simulink model "Simscape"  (R2021b)
(part 3 of 40)

  Transform37 : sm_lib/Frames and Transforms/Rigid Transform  TranslationMethod=Cartesian  TranslationStandardOffset=0  TranslationLengthUnit=mm  TranslationStandardAxis=+Z  TranslationCartesianOffset=smiData.RigidTransform(259).translation  TranslationROffset=0  TranslationROffsetUnits=m  TranslationZOffset=0  TranslationZOffsetUnits=m  TranslationThetaOffset=0  TranslationThetaOffsetUnits=deg  RotationMethod=ArbitraryAxis  RotationAngleUnits=rad  RotationStandardAxis=+Z  RotationAngle=smiData.RigidTransform(259).angle  RotationArbitraryAxis=smiData.RigidTransform(259).axis  FollAlignAxisA=+X  BaseAlignAxisA=+Y  FollAlignAxisB=+Y  BaseAlignAxisB=+Z  RotationSequenceAxes=FollowerAxes  RotationSequence=XYX  RotationSequenceAngles=[0 0 0]  RotationSequenceAnglesUnits=deg  RotationMatrix=[1 0 0; 0 1 0; 0 0 1]
  Transform38 : sm_lib/Frames and Transforms/Rigid Transform  TranslationMethod=Cartesian  TranslationStandardOffset=0  TranslationLengthUnit=mm  TranslationStandardAxis=+Z  TranslationCartesianOffset=smiData.RigidTransform(260).translation  TranslationROffset=0  TranslationROffsetUnits=m  TranslationZOffset=0  TranslationZOffsetUnits=m  TranslationThetaOffset=0  TranslationThetaOffsetUnits=deg  RotationMethod=ArbitraryAxis  RotationAngleUnits=rad  RotationStandardAxis=+Z  RotationAngle=smiData.RigidTransform(260).angle  RotationArbitraryAxis=smiData.RigidTransform(260).axis  FollAlignAxisA=+X  BaseAlignAxisA=+Y  FollAlignAxisB=+Y  BaseAlignAxisB=+Z  RotationSequenceAxes=FollowerAxes  RotationSequence=XYX  RotationSequenceAngles=[0 0 0]  RotationSequenceAnglesUnits=deg  RotationMatrix=[1 0 0; 0 1 0; 0 0 1]
  Transform39 : sm_lib/Frames and Transforms/Rigid Transform  TranslationMethod=Cartesian  TranslationStandardOffset=0  TranslationLengthUnit=mm  TranslationStandardAxis=+Z  TranslationCartesianOffset=smiData.RigidTransform(261).translation  TranslationROffset=0  TranslationROffsetUnits=m  TranslationZOffset=0  TranslationZOffsetUnits=m  TranslationThetaOffset=0  TranslationThetaOffsetUnits=deg  RotationMethod=ArbitraryAxis  RotationAngleUnits=rad  RotationStandardAxis=+Z  RotationAngle=smiData.RigidTransform(261).angle  RotationArbitraryAxis=smiData.RigidTransform(261).axis  FollAlignAxisA=+X  BaseAlignAxisA=+Y  FollAlignAxisB=+Y  BaseAlignAxisB=+Z  RotationSequenceAxes=FollowerAxes  RotationSequence=XYX  RotationSequenceAngles=[0 0 0]  RotationSequenceAnglesUnits=deg  RotationMatrix=[1 0 0; 0 1 0; 0 0 1]
  Transform4 : sm_lib/Frames and Transforms/Rigid Transform  TranslationMethod=Cartesian  TranslationStandardOffset=0  TranslationLengthUnit=mm  TranslationStandardAxis=+Z  TranslationCartesianOffset=smiData.RigidTransform(226).translation  TranslationROffset=0  TranslationROffsetUnits=m  TranslationZOffset=0  TranslationZOffsetUnits=m  TranslationThetaOffset=0  TranslationThetaOffsetUnits=deg  RotationMethod=ArbitraryAxis  RotationAngleUnits=rad  RotationStandardAxis=+Z  RotationAngle=smiData.RigidTransform(226).angle  RotationArbitraryAxis=smiData.RigidTransform(226).axis  FollAlignAxisA=+X  BaseAlignAxisA=+Y  FollAlignAxisB=+Y  BaseAlignAxisB=+Z  RotationSequenceAxes=FollowerAxes  RotationSequence=XYX  RotationSequenceAngles=[0 0 0]  RotationSequenceAnglesUnits=deg  RotationMatrix=[1 0 0; 0 1 0; 0 0 1]
  Transform40 : sm_lib/Frames and Transforms/Rigid Transform  TranslationMethod=Cartesian  TranslationStandardOffset=0  TranslationLengthUnit=mm  TranslationStandardAxis=+Z  TranslationCartesianOffset=smiData.RigidTransform(262).translation  TranslationROffset=0  TranslationROffsetUnits=m  TranslationZOffset=0  TranslationZOffsetUnits=m  TranslationThetaOffset=0  TranslationThetaOffsetUnits=deg  RotationMethod=ArbitraryAxis  RotationAngleUnits=rad  RotationStandardAxis=+Z  RotationAngle=smiData.RigidTransform(262).angle  RotationArbitraryAxis=smiData.RigidTransform(262).axis  FollAlignAxisA=+X  BaseAlignAxisA=+Y  FollAlignAxisB=+Y  BaseAlignAxisB=+Z  RotationSequenceAxes=FollowerAxes  RotationSequence=XYX  RotationSequenceAngles=[0 0 0]  RotationSequenceAnglesUnits=deg  RotationMatrix=[1 0 0; 0 1 0; 0 0 1]
  Transform41 : sm_lib/Frames and Transforms/Rigid Transform  TranslationMethod=Cartesian  TranslationStandardOffset=0  TranslationLengthUnit=mm  TranslationStandardAxis=+Z  TranslationCartesianOffset=smiData.RigidTransform(263).translation  TranslationROffset=0  TranslationROffsetUnits=m  TranslationZOffset=0  TranslationZOffsetUnits=m  TranslationThetaOffset=0  TranslationThetaOffsetUnits=deg  RotationMethod=ArbitraryAxis  RotationAngleUnits=rad  RotationStandardAxis=+Z  RotationAngle=smiData.RigidTransform(263).angle  RotationArbitraryAxis=smiData.RigidTransform(263).axis  FollAlignAxisA=+X  BaseAlignAxisA=+Y  FollAlignAxisB=+Y  BaseAlignAxisB=+Z  RotationSequenceAxes=FollowerAxes  RotationSequence=XYX  RotationSequenceAngles=[0 0 0]  RotationSequenceAnglesUnits=deg  RotationMatrix=[1 0 0; 0 1 0; 0 0 1]
  Transform42 : sm_lib/Frames and Transforms/Rigid Transform  TranslationMethod=Cartesian  TranslationStandardOffset=0  TranslationLengthUnit=mm  TranslationStandardAxis=+Z  TranslationCartesianOffset=smiData.RigidTransform(264).translation  TranslationROffset=0  TranslationROffsetUnits=m  TranslationZOffset=0  TranslationZOffsetUnits=m  TranslationThetaOffset=0  TranslationThetaOffsetUnits=deg  RotationMethod=ArbitraryAxis  RotationAngleUnits=rad  RotationStandardAxis=+Z  RotationAngle=smiData.RigidTransform(264).angle  RotationArbitraryAxis=smiData.RigidTransform(264).axis  FollAlignAxisA=+X  BaseAlignAxisA=+Y  FollAlignAxisB=+Y  BaseAlignAxisB=+Z  RotationSequenceAxes=FollowerAxes  RotationSequence=XYX  RotationSequenceAngles=[0 0 0]  RotationSequenceAnglesUnits=deg  RotationMatrix=[1 0 0; 0 1 0; 0 0 1]
  Transform43 : sm_lib/Frames and Transforms/Rigid Transform  TranslationMethod=Cartesian  TranslationStandardOffset=0  TranslationLengthUnit=mm  TranslationStandardAxis=+Z  TranslationCartesianOffset=smiData.RigidTransform(265).translation  TranslationROffset=0  TranslationROffsetUnits=m  TranslationZOffset=0  TranslationZOffsetUnits=m  TranslationThetaOffset=0  TranslationThetaOffsetUnits=deg  RotationMethod=ArbitraryAxis  RotationAngleUnits=rad  RotationStandardAxis=+Z  RotationAngle=smiData.RigidTransform(265).angle  RotationArbitraryAxis=smiData.RigidTransform(265).axis  FollAlignAxisA=+X  BaseAlignAxisA=+Y  FollAlignAxisB=+Y  BaseAlignAxisB=+Z  RotationSequenceAxes=FollowerAxes  RotationSequence=XYX  RotationSequenceAngles=[0 0 0]  RotationSequenceAnglesUnits=deg  RotationMatrix=[1 0 0; 0 1 0; 0 0 1]
  Transform44 : sm_lib/Frames and Transforms/Rigid Transform  TranslationMethod=Cartesian  TranslationStandardOffset=0  TranslationLengthUnit=mm  TranslationStandardAxis=+Z  TranslationCartesianOffset=smiData.RigidTransform(266).translation  TranslationROffset=0  TranslationROffsetUnits=m  TranslationZOffset=0  TranslationZOffsetUnits=m  TranslationThetaOffset=0  TranslationThetaOffsetUnits=deg  RotationMethod=ArbitraryAxis  RotationAngleUnits=rad  RotationStandardAxis=+Z  RotationAngle=smiData.RigidTransform(266).angle  RotationArbitraryAxis=smiData.RigidTransform(266).axis  FollAlignAxisA=+X  BaseAlignAxisA=+Y  FollAlignAxisB=+Y  BaseAlignAxisB=+Z  RotationSequenceAxes=FollowerAxes  RotationSequence=XYX  RotationSequenceAngles=[0 0 0]  RotationSequenceAnglesUnits=deg  RotationMatrix=[1 0 0; 0 1 0; 0 0 1]
  Transform45 : sm_lib/Frames and Transforms/Rigid Transform  TranslationMethod=Cartesian  TranslationStandardOffset=0  TranslationLengthUnit=mm  TranslationStandardAxis=+Z  TranslationCartesianOffset=smiData.RigidTransform(267).translation  TranslationROffset=0  TranslationROffsetUnits=m  TranslationZOffset=0  TranslationZOffsetUnits=m  TranslationThetaOffset=0  TranslationThetaOffsetUnits=deg  RotationMethod=ArbitraryAxis  RotationAngleUnits=rad  RotationStandardAxis=+Z  RotationAngle=smiData.RigidTransform(267).angle  RotationArbitraryAxis=smiData.RigidTransform(267).axis  FollAlignAxisA=+X  BaseAlignAxisA=+Y  FollAlignAxisB=+Y  BaseAlignAxisB=+Z  RotationSequenceAxes=FollowerAxes  RotationSequence=XYX  RotationSequenceAngles=[0 0 0]  RotationSequenceAnglesUnits=deg  RotationMatrix=[1 0 0; 0 1 0; 0 0 1]
  Transform46 : sm_lib/Frames and Transforms/Rigid Transform  TranslationMethod=Cartesian  TranslationStandardOffset=0  TranslationLengthUnit=mm  TranslationStandardAxis=+Z  TranslationCartesianOffset=smiData.RigidTransform(268).translation  TranslationROffset=0  TranslationROffsetUnits=m  TranslationZOffset=0  TranslationZOffsetUnits=m  TranslationThetaOffset=0  TranslationThetaOffsetUnits=deg  RotationMethod=ArbitraryAxis  RotationAngleUnits=rad  RotationStandardAxis=+Z  RotationAngle=smiData.RigidTransform(268).angle  RotationArbitraryAxis=smiData.RigidTransform(268).axis  FollAlignAxisA=+X  BaseAlignAxisA=+Y  FollAlignAxisB=+Y  BaseAlignAxisB=+Z  RotationSequenceAxes=FollowerAxes  RotationSequence=XYX  RotationSequenceAngles=[0 0 0]  RotationSequenceAnglesUnits=deg  RotationMatrix=[1 0 0; 0 1 0; 0 0 1]
  Transform47 : sm_lib/Frames and Transforms/Rigid Transform  TranslationMethod=Cartesian  TranslationStandardOffset=0  TranslationLengthUnit=mm  TranslationStandardAxis=+Z  TranslationCartesianOffset=smiData.RigidTransform(269).translation  TranslationROffset=0  TranslationROffsetUnits=m  TranslationZOffset=0  TranslationZOffsetUnits=m  TranslationThetaOffset=0  TranslationThetaOffsetUnits=deg  RotationMethod=ArbitraryAxis  RotationAngleUnits=rad  RotationStandardAxis=+Z  RotationAngle=smiData.RigidTransform(269).angle  RotationArbitraryAxis=smiData.RigidTransform(269).axis  FollAlignAxisA=+X  BaseAlignAxisA=+Y  FollAlignAxisB=+Y  BaseAlignAxisB=+Z  RotationSequenceAxes=FollowerAxes  RotationSequence=XYX  RotationSequenceAngles=[0 0 0]  RotationSequenceAnglesUnits=deg  RotationMatrix=[1 0 0; 0 1 0; 0 0 1]
  Transform48 : sm_lib/Frames and Transforms/Rigid Transform  TranslationMethod=Cartesian  TranslationStandardOffset=0  TranslationLengthUnit=mm  TranslationStandardAxis=+Z  TranslationCartesianOffset=smiData.RigidTransform(270).translation  TranslationROffset=0  TranslationROffsetUnits=m  TranslationZOffset=0  TranslationZOffsetUnits=m  TranslationThetaOffset=0  TranslationThetaOffsetUnits=deg  RotationMethod=ArbitraryAxis  RotationAngleUnits=rad  RotationStandardAxis=+Z  RotationAngle=smiData.RigidTransform(270).angle  RotationArbitraryAxis=smiData.RigidTransform(270).axis  FollAlignAxisA=+X  BaseAlignAxisA=+Y  FollAlignAxisB=+Y  BaseAlignAxisB=+Z  RotationSequenceAxes=FollowerAxes  RotationSequence=XYX  RotationSequenceAngles=[0 0 0]  RotationSequenceAnglesUnits=deg  RotationMatrix=[1 0 0; 0 1 0; 0 0 1]
  Transform49 : sm_lib/Frames and Transforms/Rigid Transform  TranslationMethod=Cartesian  TranslationStandardOffset=0  TranslationLengthUnit=mm  TranslationStandardAxis=+Z  TranslationCartesianOffset=smiData.RigidTransform(271).translation  TranslationROffset=0  TranslationROffsetUnits=m  TranslationZOffset=0  TranslationZOffsetUnits=m  TranslationThetaOffset=0  TranslationThetaOffsetUnits=deg  RotationMethod=ArbitraryAxis  RotationAngleUnits=rad  RotationStandardAxis=+Z  RotationAngle=smiData.RigidTransform(271).angle  RotationArbitraryAxis=smiData.RigidTransform(271).axis  FollAlignAxisA=+X  BaseAlignAxisA=+Y  FollAlignAxisB=+Y  BaseAlignAxisB=+Z  RotationSequenceAxes=FollowerAxes  RotationSequence=XYX  RotationSequenceAngles=[0 0 0]  RotationSequenceAnglesUnits=deg  RotationMatrix=[1 0 0; 0 1 0; 0 0 1]
  Transform5 : sm_lib/Frames and Transforms/Rigid Transform  TranslationMethod=Cartesian  TranslationStandardOffset=0  TranslationLengthUnit=mm  TranslationStandardAxis=+Z  TranslationCartesianOffset=smiData.RigidTransform(227).translation  TranslationROffset=0  TranslationROffsetUnits=m  TranslationZOffset=0  TranslationZOffsetUnits=m  TranslationThetaOffset=0  TranslationThetaOffsetUnits=deg  RotationMethod=ArbitraryAxis  RotationAngleUnits=rad  RotationStandardAxis=+Z  RotationAngle=smiData.RigidTransform(227).angle  RotationArbitraryAxis=smiData.RigidTransform(227).axis  FollAlignAxisA=+X  BaseAlignAxisA=+Y  FollAlignAxisB=+Y  BaseAlignAxisB=+Z  RotationSequenceAxes=FollowerAxes  RotationSequence=XYX  RotationSequenceAngles=[0 0 0]  RotationSequenceAnglesUnits=deg  RotationMatrix=[1 0 0; 0 1 0; 0 0 1]
  Transform50 : sm_lib/Frames and Transforms/Rigid Transform  TranslationMethod=Cartesian  TranslationStandardOffset=0  TranslationLengthUnit=mm  TranslationStandardAxis=+Z  TranslationCartesianOffset=smiData.RigidTransform(272).translation  TranslationROffset=0  TranslationROffsetUnits=m  TranslationZOffset=0  TranslationZOffsetUnits=m  TranslationThetaOffset=0  TranslationThetaOffsetUnits=deg  RotationMethod=ArbitraryAxis  RotationAngleUnits=rad  RotationStandardAxis=+Z  RotationAngle=smiData.RigidTransform(272).angle  RotationArbitraryAxis=smiData.RigidTransform(272).axis  FollAlignAxisA=+X  BaseAlignAxisA=+Y  FollAlignAxisB=+Y  BaseAlignAxisB=+Z  RotationSequenceAxes=FollowerAxes  RotationSequence=XYX  RotationSequenceAngles=[0 0 0]  RotationSequenceAnglesUnits=deg  RotationMatrix=[1 0 0; 0 1 0; 0 0 1]
  Transform51 : sm_lib/Frames and Transforms/Rigid Transform  TranslationMethod=Cartesian  TranslationStandardOffset=0  TranslationLengthUnit=mm  TranslationStandardAxis=+Z  TranslationCartesianOffset=smiData.RigidTransform(273).translation  TranslationROffset=0  TranslationROffsetUnits=m  TranslationZOffset=0  TranslationZOffsetUnits=m  TranslationThetaOffset=0  TranslationThetaOffsetUnits=deg  RotationMethod=ArbitraryAxis  RotationAngleUnits=rad  RotationStandardAxis=+Z  RotationAngle=smiData.RigidTransform(273).angle  RotationArbitraryAxis=smiData.RigidTransform(273).axis  FollAlignAxisA=+X  BaseAlignAxisA=+Y  FollAlignAxisB=+Y  BaseAlignAxisB=+Z  RotationSequenceAxes=FollowerAxes  RotationSequence=XYX  RotationSequenceAngles=[0 0 0]  RotationSequenceAnglesUnits=deg  RotationMatrix=[1 0 0; 0 1 0; 0 0 1]
  Transform52 : sm_lib/Frames and Transforms/Rigid Transform  TranslationMethod=Cartesian  TranslationStandardOffset=0  TranslationLengthUnit=mm  TranslationStandardAxis=+Z  TranslationCartesianOffset=smiData.RigidTransform(274).translation  TranslationROffset=0  TranslationROffsetUnits=m  TranslationZOffset=0  TranslationZOffsetUnits=m  TranslationThetaOffset=0  TranslationThetaOffsetUnits=deg  RotationMethod=ArbitraryAxis  RotationAngleUnits=rad  RotationStandardAxis=+Z  RotationAngle=smiData.RigidTransform(274).angle  RotationArbitraryAxis=smiData.RigidTransform(274).axis  FollAlignAxisA=+X  BaseAlignAxisA=+Y  FollAlignAxisB=+Y  BaseAlignAxisB=+Z  RotationSequenceAxes=FollowerAxes  RotationSequence=XYX  RotationSequenceAngles=[0 0 0]  RotationSequenceAnglesUnits=deg  RotationMatrix=[1 0 0; 0 1 0; 0 0 1]
  Transform53 : sm_lib/Frames and Transforms/Rigid Transform  TranslationMethod=Cartesian  TranslationStandardOffset=0  TranslationLengthUnit=mm  TranslationStandardAxis=+Z  TranslationCartesianOffset=smiData.RigidTransform(275).translation  TranslationROffset=0  TranslationROffsetUnits=m  TranslationZOffset=0  TranslationZOffsetUnits=m  TranslationThetaOffset=0  TranslationThetaOffsetUnits=deg  RotationMethod=ArbitraryAxis  RotationAngleUnits=rad  RotationStandardAxis=+Z  RotationAngle=smiData.RigidTransform(275).angle  RotationArbitraryAxis=smiData.RigidTransform(275).axis  FollAlignAxisA=+X  BaseAlignAxisA=+Y  FollAlignAxisB=+Y  BaseAlignAxisB=+Z  RotationSequenceAxes=FollowerAxes  RotationSequence=XYX  RotationSequenceAngles=[0 0 0]  RotationSequenceAnglesUnits=deg  RotationMatrix=[1 0 0; 0 1 0; 0 0 1]
  Transform54 : sm_lib/Frames and Transforms/Rigid Transform  TranslationMethod=Cartesian  TranslationStandardOffset=0  TranslationLengthUnit=mm  TranslationStandardAxis=+Z  TranslationCartesianOffset=smiData.RigidTransform(276).translation  TranslationROffset=0  TranslationROffsetUnits=m  TranslationZOffset=0  TranslationZOffsetUnits=m  TranslationThetaOffset=0  TranslationThetaOffsetUnits=deg  RotationMethod=ArbitraryAxis  RotationAngleUnits=rad  RotationStandardAxis=+Z  RotationAngle=smiData.RigidTransform(276).angle  RotationArbitraryAxis=smiData.RigidTransform(276).axis  FollAlignAxisA=+X  BaseAlignAxisA=+Y  FollAlignAxisB=+Y  BaseAlignAxisB=+Z  RotationSequenceAxes=FollowerAxes  RotationSequence=XYX  RotationSequenceAngles=[0 0 0]  RotationSequenceAnglesUnits=deg  RotationMatrix=[1 0 0; 0 1 0; 0 0 1]
  Transform55 : sm_lib/Frames and Transforms/Rigid Transform  TranslationMethod=Cartesian  TranslationStandardOffset=0  TranslationLengthUnit=mm  TranslationStandardAxis=+Z  TranslationCartesianOffset=smiData.RigidTransform(277).translation  TranslationROffset=0  TranslationROffsetUnits=m  TranslationZOffset=0  TranslationZOffsetUnits=m  TranslationThetaOffset=0  TranslationThetaOffsetUnits=deg  RotationMethod=ArbitraryAxis  RotationAngleUnits=rad  RotationStandardAxis=+Z  RotationAngle=smiData.RigidTransform(277).angle  RotationArbitraryAxis=smiData.RigidTransform(277).axis  FollAlignAxisA=+X  BaseAlignAxisA=+Y  FollAlignAxisB=+Y  BaseAlignAxisB=+Z  RotationSequenceAxes=FollowerAxes  RotationSequence=XYX  RotationSequenceAngles=[0 0 0]  RotationSequenceAnglesUnits=deg  RotationMatrix=[1 0 0; 0 1 0; 0 0 1]
  Transform56 : sm_lib/Frames and Transforms/Rigid Transform  TranslationMethod=Cartesian  TranslationStandardOffset=0  TranslationLengthUnit=mm  TranslationStandardAxis=+Z  TranslationCartesianOffset=smiData.RigidTransform(278).translation  TranslationROffset=0  TranslationROffsetUnits=m  TranslationZOffset=0  TranslationZOffsetUnits=m  TranslationThetaOffset=0  TranslationThetaOffsetUnits=deg  RotationMethod=ArbitraryAxis  RotationAngleUnits=rad  RotationStandardAxis=+Z  RotationAngle=smiData.RigidTransform(278).angle  RotationArbitraryAxis=smiData.RigidTransform(278).axis  FollAlignAxisA=+X  BaseAlignAxisA=+Y  FollAlignAxisB=+Y  BaseAlignAxisB=+Z  RotationSequenceAxes=FollowerAxes  RotationSequence=XYX  RotationSequenceAngles=[0 0 0]  RotationSequenceAnglesUnits=deg  RotationMatrix=[1 0 0; 0 1 0; 0 0 1]
  Transform57 : sm_lib/Frames and Transforms/Rigid Transform  TranslationMethod=Cartesian  TranslationStandardOffset=0  TranslationLengthUnit=mm  TranslationStandardAxis=+Z  TranslationCartesianOffset=smiData.RigidTransform(279).translation  TranslationROffset=0  TranslationROffsetUnits=m  TranslationZOffset=0  TranslationZOffsetUnits=m  TranslationThetaOffset=0  TranslationThetaOffsetUnits=deg  RotationMethod=ArbitraryAxis  RotationAngleUnits=rad  RotationStandardAxis=+Z  RotationAngle=smiData.RigidTransform(279).angle  RotationArbitraryAxis=smiData.RigidTransform(279).axis  FollAlignAxisA=+X  BaseAlignAxisA=+Y  FollAlignAxisB=+Y  BaseAlignAxisB=+Z  RotationSequenceAxes=FollowerAxes  RotationSequence=XYX  RotationSequenceAngles=[0 0 0]  RotationSequenceAnglesUnits=deg  RotationMatrix=[1 0 0; 0 1 0; 0 0 1]
  Transform58 : sm_lib/Frames and Transforms/Rigid Transform  TranslationMethod=Cartesian  TranslationStandardOffset=0  TranslationLengthUnit=mm  TranslationStandardAxis=+Z  TranslationCartesianOffset=smiData.RigidTransform(280).translation  TranslationROffset=0  TranslationROffsetUnits=m  TranslationZOffset=0  TranslationZOffsetUnits=m  TranslationThetaOffset=0  TranslationThetaOffsetUnits=deg  RotationMethod=ArbitraryAxis  RotationAngleUnits=rad  RotationStandardAxis=+Z  RotationAngle=smiData.RigidTransform(280).angle  RotationArbitraryAxis=smiData.RigidTransform(280).axis  FollAlignAxisA=+X  BaseAlignAxisA=+Y  FollAlignAxisB=+Y  BaseAlignAxisB=+Z  RotationSequenceAxes=FollowerAxes  RotationSequence=XYX  RotationSequenceAngles=[0 0 0]  RotationSequenceAnglesUnits=deg  RotationMatrix=[1 0 0; 0 1 0; 0 0 1]
  Transform59 : sm_lib/Frames and Transforms/Rigid Transform  TranslationMethod=Cartesian  TranslationStandardOffset=0  TranslationLengthUnit=mm  TranslationStandardAxis=+Z  TranslationCartesianOffset=smiData.RigidTransform(281).translation  TranslationROffset=0  TranslationROffsetUnits=m  TranslationZOffset=0  TranslationZOffsetUnits=m  TranslationThetaOffset=0  TranslationThetaOffsetUnits=deg  RotationMethod=ArbitraryAxis  RotationAngleUnits=rad  RotationStandardAxis=+Z  RotationAngle=smiData.RigidTransform(281).angle  RotationArbitraryAxis=smiData.RigidTransform(281).axis  FollAlignAxisA=+X  BaseAlignAxisA=+Y  FollAlignAxisB=+Y  BaseAlignAxisB=+Z  RotationSequenceAxes=FollowerAxes  RotationSequence=XYX  RotationSequenceAngles=[0 0 0]  RotationSequenceAnglesUnits=deg  RotationMatrix=[1 0 0; 0 1 0; 0 0 1]
  Transform6 : sm_lib/Frames and Transforms/Rigid Transform  TranslationMethod=Cartesian  TranslationStandardOffset=0  TranslationLengthUnit=mm  TranslationStandardAxis=+Z  TranslationCartesianOffset=smiData.RigidTransform(228).translation  TranslationROffset=0  TranslationROffsetUnits=m  TranslationZOffset=0  TranslationZOffsetUnits=m  TranslationThetaOffset=0  TranslationThetaOffsetUnits=deg  RotationMethod=ArbitraryAxis  RotationAngleUnits=rad  RotationStandardAxis=+Z  RotationAngle=smiData.RigidTransform(228).angle  RotationArbitraryAxis=smiData.RigidTransform(228).axis  FollAlignAxisA=+X  BaseAlignAxisA=+Y  FollAlignAxisB=+Y  BaseAlignAxisB=+Z  RotationSequenceAxes=FollowerAxes  RotationSequence=XYX  RotationSequenceAngles=[0 0 0]  RotationSequenceAnglesUnits=deg  RotationMatrix=[1 0 0; 0 1 0; 0 0 1]
  Transform60 : sm_lib/Frames and Transforms/Rigid Transform  TranslationMethod=Cartesian  TranslationStandardOffset=0  TranslationLengthUnit=mm  TranslationStandardAxis=+Z  TranslationCartesianOffset=smiData.RigidTransform(282).translation  TranslationROffset=0  TranslationROffsetUnits=m  TranslationZOffset=0  TranslationZOffsetUnits=m  TranslationThetaOffset=0  TranslationThetaOffsetUnits=deg  RotationMethod=ArbitraryAxis  RotationAngleUnits=rad  RotationStandardAxis=+Z  RotationAngle=smiData.RigidTransform(282).angle  RotationArbitraryAxis=smiData.RigidTransform(282).axis  FollAlignAxisA=+X  BaseAlignAxisA=+Y  FollAlignAxisB=+Y  BaseAlignAxisB=+Z  RotationSequenceAxes=FollowerAxes  RotationSequence=XYX  RotationSequenceAngles=[0 0 0]  RotationSequenceAnglesUnits=deg  RotationMatrix=[1 0 0; 0 1 0; 0 0 1]
  Transform61 : sm_lib/Frames and Transforms/Rigid Transform  TranslationMethod=Cartesian  TranslationStandardOffset=0  TranslationLengthUnit=mm  TranslationStandardAxis=+Z  TranslationCartesianOffset=smiData.RigidTransform(283).translation  TranslationROffset=0  TranslationROffsetUnits=m  TranslationZOffset=0  TranslationZOffsetUnits=m  TranslationThetaOffset=0  TranslationThetaOffsetUnits=deg  RotationMethod=ArbitraryAxis  RotationAngleUnits=rad  RotationStandardAxis=+Z  RotationAngle=smiData.RigidTransform(283).angle  RotationArbitraryAxis=smiData.RigidTransform(283).axis  FollAlignAxisA=+X  BaseAlignAxisA=+Y  FollAlignAxisB=+Y  BaseAlignAxisB=+Z  RotationSequenceAxes=FollowerAxes  RotationSequence=XYX  RotationSequenceAngles=[0 0 0]  RotationSequenceAnglesUnits=deg  RotationMatrix=[1 0 0; 0 1 0; 0 0 1]
  Transform62 : sm_lib/Frames and Transforms/Rigid Transform  TranslationMethod=Cartesian  TranslationStandardOffset=0  TranslationLengthUnit=mm  TranslationStandardAxis=+Z  TranslationCartesianOffset=smiData.RigidTransform(284).translation  TranslationROffset=0  TranslationROffsetUnits=m  TranslationZOffset=0  TranslationZOffsetUnits=m  TranslationThetaOffset=0  TranslationThetaOffsetUnits=deg  RotationMethod=ArbitraryAxis  RotationAngleUnits=rad  RotationStandardAxis=+Z  RotationAngle=smiData.RigidTransform(284).angle  RotationArbitraryAxis=smiData.RigidTransform(284).axis  FollAlignAxisA=+X  BaseAlignAxisA=+Y  FollAlignAxisB=+Y  BaseAlignAxisB=+Z  RotationSequenceAxes=FollowerAxes  RotationSequence=XYX  RotationSequenceAngles=[0 0 0]  RotationSequenceAnglesUnits=deg  RotationMatrix=[1 0 0; 0 1 0; 0 0 1]
  Transform63 : sm_lib/Frames and Transforms/Rigid Transform  TranslationMethod=Cartesian  TranslationStandardOffset=0  TranslationLengthUnit=mm  TranslationStandardAxis=+Z  TranslationCartesianOffset=smiData.RigidTransform(285).translation  TranslationROffset=0  TranslationROffsetUnits=m  TranslationZOffset=0  TranslationZOffsetUnits=m  TranslationThetaOffset=0  TranslationThetaOffsetUnits=deg  RotationMethod=ArbitraryAxis  RotationAngleUnits=rad  RotationStandardAxis=+Z  RotationAngle=smiData.RigidTransform(285).angle  RotationArbitraryAxis=smiData.RigidTransform(285).axis  FollAlignAxisA=+X  BaseAlignAxisA=+Y  FollAlignAxisB=+Y  BaseAlignAxisB=+Z  RotationSequenceAxes=FollowerAxes  RotationSequence=XYX  RotationSequenceAngles=[0 0 0]  RotationSequenceAnglesUnits=deg  RotationMatrix=[1 0 0; 0 1 0; 0 0 1]
  Transform64 : sm_lib/Frames and Transforms/Rigid Transform  TranslationMethod=Cartesian  TranslationStandardOffset=0  TranslationLengthUnit=mm  TranslationStandardAxis=+Z  TranslationCartesianOffset=smiData.RigidTransform(286).translation  TranslationROffset=0  TranslationROffsetUnits=m  TranslationZOffset=0  TranslationZOffsetUnits=m  TranslationThetaOffset=0  TranslationThetaOffsetUnits=deg  RotationMethod=ArbitraryAxis  RotationAngleUnits=rad  RotationStandardAxis=+Z  RotationAngle=smiData.RigidTransform(286).angle  RotationArbitraryAxis=smiData.RigidTransform(286).axis  FollAlignAxisA=+X  BaseAlignAxisA=+Y  FollAlignAxisB=+Y  BaseAlignAxisB=+Z  RotationSequenceAxes=FollowerAxes  RotationSequence=XYX  RotationSequenceAngles=[0 0 0]  RotationSequenceAnglesUnits=deg  RotationMatrix=[1 0 0; 0 1 0; 0 0 1]
  Transform65 : sm_lib/Frames and Transforms/Rigid Transform  TranslationMethod=Cartesian  TranslationStandardOffset=0  TranslationLengthUnit=mm  TranslationStandardAxis=+Z  TranslationCartesianOffset=smiData.RigidTransform(287).translation  TranslationROffset=0  TranslationROffsetUnits=m  TranslationZOffset=0  TranslationZOffsetUnits=m  TranslationThetaOffset=0  TranslationThetaOffsetUnits=deg  RotationMethod=ArbitraryAxis  RotationAngleUnits=rad  RotationStandardAxis=+Z  RotationAngle=smiData.RigidTransform(287).angle  RotationArbitraryAxis=smiData.RigidTransform(287).axis  FollAlignAxisA=+X  BaseAlignAxisA=+Y  FollAlignAxisB=+Y  BaseAlignAxisB=+Z  RotationSequenceAxes=FollowerAxes  RotationSequence=XYX  RotationSequenceAngles=[0 0 0]  RotationSequenceAnglesUnits=deg  RotationMatrix=[1 0 0; 0 1 0; 0 0 1]
  Transform66 : sm_lib/Frames and Transforms/Rigid Transform  TranslationMethod=Cartesian  TranslationStandardOffset=0  TranslationLengthUnit=mm  TranslationStandardAxis=+Z  TranslationCartesianOffset=smiData.RigidTransform(288).translation  TranslationROffset=0  TranslationROffsetUnits=m  TranslationZOffset=0  TranslationZOffsetUnits=m  TranslationThetaOffset=0  TranslationThetaOffsetUnits=deg  RotationMethod=ArbitraryAxis  RotationAngleUnits=rad  RotationStandardAxis=+Z  RotationAngle=smiData.RigidTransform(288).angle  RotationArbitraryAxis=smiData.RigidTransform(288).axis  FollAlignAxisA=+X  BaseAlignAxisA=+Y  FollAlignAxisB=+Y  BaseAlignAxisB=+Z  RotationSequenceAxes=FollowerAxes  RotationSequence=XYX  RotationSequenceAngles=[0 0 0]  RotationSequenceAnglesUnits=deg  RotationMatrix=[1 0 0; 0 1 0; 0 0 1]
  Transform67 : sm_lib/Frames and Transforms/Rigid Transform  TranslationMethod=Cartesian  TranslationStandardOffset=0  TranslationLengthUnit=mm  TranslationStandardAxis=+Z  TranslationCartesianOffset=smiData.RigidTransform(289).translation  TranslationROffset=0  TranslationROffsetUnits=m  TranslationZOffset=0  TranslationZOffsetUnits=m  TranslationThetaOffset=0  TranslationThetaOffsetUnits=deg  RotationMethod=ArbitraryAxis  RotationAngleUnits=rad  RotationStandardAxis=+Z  RotationAngle=smiData.RigidTransform(289).angle  RotationArbitraryAxis=smiData.RigidTransform(289).axis  FollAlignAxisA=+X  BaseAlignAxisA=+Y  FollAlignAxisB=+Y  BaseAlignAxisB=+Z  RotationSequenceAxes=FollowerAxes  RotationSequence=XYX  RotationSequenceAngles=[0 0 0]  RotationSequenceAnglesUnits=deg  RotationMatrix=[1 0 0; 0 1 0; 0 0 1]
  Transform68 : sm_lib/Frames and Transforms/Rigid Transform  TranslationMethod=Cartesian  TranslationStandardOffset=0  TranslationLengthUnit=mm  TranslationStandardAxis=+Z  TranslationCartesianOffset=smiData.RigidTransform(290).translation  TranslationROffset=0  TranslationROffsetUnits=m  TranslationZOffset=0  TranslationZOffsetUnits=m  TranslationThetaOffset=0  TranslationThetaOffsetUnits=deg  RotationMethod=ArbitraryAxis  RotationAngleUnits=rad  RotationStandardAxis=+Z  RotationAngle=smiData.RigidTransform(290).angle  RotationArbitraryAxis=smiData.RigidTransform(290).axis  FollAlignAxisA=+X  BaseAlignAxisA=+Y  FollAlignAxisB=+Y  BaseAlignAxisB=+Z  RotationSequenceAxes=FollowerAxes  RotationSequence=XYX  RotationSequenceAngles=[0 0 0]  RotationSequenceAnglesUnits=deg  RotationMatrix=[1 0 0; 0 1 0; 0 0 1]
  Transform69 : sm_lib/Frames and Transforms/Rigid Transform  TranslationMethod=Cartesian  TranslationStandardOffset=0  TranslationLengthUnit=mm  TranslationStandardAxis=+Z  TranslationCartesianOffset=smiData.RigidTransform(291).translation  TranslationROffset=0  TranslationROffsetUnits=m  TranslationZOffset=0  TranslationZOffsetUnits=m  TranslationThetaOffset=0  TranslationThetaOffsetUnits=deg  RotationMethod=ArbitraryAxis  RotationAngleUnits=rad  RotationStandardAxis=+Z  RotationAngle=smiData.RigidTransform(291).angle  RotationArbitraryAxis=smiData.RigidTransform(291).axis  FollAlignAxisA=+X  BaseAlignAxisA=+Y  FollAlignAxisB=+Y  BaseAlignAxisB=+Z  RotationSequenceAxes=FollowerAxes  RotationSequence=XYX  RotationSequenceAngles=[0 0 0]  RotationSequenceAnglesUnits=deg  RotationMatrix=[1 0 0; 0 1 0; 0 0 1]
  Transform7 : sm_lib/Frames and Transforms/Rigid Transform  TranslationMethod=Cartesian  TranslationStandardOffset=0  TranslationLengthUnit=mm  TranslationStandardAxis=+Z  TranslationCartesianOffset=smiData.RigidTransform(229).translation  TranslationROffset=0  TranslationROffsetUnits=m  TranslationZOffset=0  TranslationZOffsetUnits=m  TranslationThetaOffset=0  TranslationThetaOffsetUnits=deg  RotationMethod=ArbitraryAxis  RotationAngleUnits=rad  RotationStandardAxis=+Z  RotationAngle=smiData.RigidTransform(229).angle  RotationArbitraryAxis=smiData.RigidTransform(229).axis  FollAlignAxisA=+X  BaseAlignAxisA=+Y  FollAlignAxisB=+Y  BaseAlignAxisB=+Z  RotationSequenceAxes=FollowerAxes  RotationSequence=XYX  RotationSequenceAngles=[0 0 0]  RotationSequenceAnglesUnits=deg  RotationMatrix=[1 0 0; 0 1 0; 0 0 1]
  Transform70 : sm_lib/Frames and Transforms/Rigid Transform  TranslationMethod=Cartesian  TranslationStandardOffset=0  TranslationLengthUnit=mm  TranslationStandardAxis=+Z  TranslationCartesianOffset=smiData.RigidTransform(292).translation  TranslationROffset=0  TranslationROffsetUnits=m  TranslationZOffset=0  TranslationZOffsetUnits=m  TranslationThetaOffset=0  TranslationThetaOffsetUnits=deg  RotationMethod=ArbitraryAxis  RotationAngleUnits=rad  RotationStandardAxis=+Z  RotationAngle=smiData.RigidTransform(292).angle  RotationArbitraryAxis=smiData.RigidTransform(292).axis  FollAlignAxisA=+X  BaseAlignAxisA=+Y  FollAlignAxisB=+Y  BaseAlignAxisB=+Z  RotationSequenceAxes=FollowerAxes  RotationSequence=XYX  RotationSequenceAngles=[0 0 0]  RotationSequenceAnglesUnits=deg  RotationMatrix=[1 0 0; 0 1 0; 0 0 1]
  Transform71 : sm_lib/Frames and Transforms/Rigid Transform  TranslationMethod=Cartesian  TranslationStandardOffset=0  TranslationLengthUnit=mm  TranslationStandardAxis=+Z  TranslationCartesianOffset=smiData.RigidTransform(293).translation  TranslationROffset=0  TranslationROffsetUnits=m  TranslationZOffset=0  TranslationZOffsetUnits=m  TranslationThetaOffset=0  TranslationThetaOffsetUnits=deg  RotationMethod=ArbitraryAxis  RotationAngleUnits=rad  RotationStandardAxis=+Z  RotationAngle=smiData.RigidTransform(293).angle  RotationArbitraryAxis=smiData.RigidTransform(293).axis  FollAlignAxisA=+X  BaseAlignAxisA=+Y  FollAlignAxisB=+Y  BaseAlignAxisB=+Z  RotationSequenceAxes=FollowerAxes  RotationSequence=XYX  RotationSequenceAngles=[0 0 0]  RotationSequenceAnglesUnits=deg  RotationMatrix=[1 0 0; 0 1 0; 0 0 1]
  Transform72 : sm_lib/Frames and Transforms/Rigid Transform  TranslationMethod=Cartesian  TranslationStandardOffset=0  TranslationLengthUnit=mm  TranslationStandardAxis=+Z  TranslationCartesianOffset=smiData.RigidTransform(294).translation  TranslationROffset=0  TranslationROffsetUnits=m  TranslationZOffset=0  TranslationZOffsetUnits=m  TranslationThetaOffset=0  TranslationThetaOffsetUnits=deg  RotationMethod=ArbitraryAxis  RotationAngleUnits=rad  RotationStandardAxis=+Z  RotationAngle=smiData.RigidTransform(294).angle  RotationArbitraryAxis=smiData.RigidTransform(294).axis  FollAlignAxisA=+X  BaseAlignAxisA=+Y  FollAlignAxisB=+Y  BaseAlignAxisB=+Z  RotationSequenceAxes=FollowerAxes  RotationSequence=XYX  RotationSequenceAngles=[0 0 0]  RotationSequenceAnglesUnits=deg  RotationMatrix=[1 0 0; 0 1 0; 0 0 1]
  Transform73 : sm_lib/Frames and Transforms/Rigid Transform  TranslationMethod=Cartesian  TranslationStandardOffset=0  TranslationLengthUnit=mm  TranslationStandardAxis=+Z  TranslationCartesianOffset=smiData.RigidTransform(295).translation  TranslationROffset=0  TranslationROffsetUnits=m  TranslationZOffset=0  TranslationZOffsetUnits=m  TranslationThetaOffset=0  TranslationThetaOffsetUnits=deg  RotationMethod=ArbitraryAxis  RotationAngleUnits=rad  RotationStandardAxis=+Z  RotationAngle=smiData.RigidTransform(295).angle  RotationArbitraryAxis=smiData.RigidTransform(295).axis  FollAlignAxisA=+X  BaseAlignAxisA=+Y  FollAlignAxisB=+Y  BaseAlignAxisB=+Z  RotationSequenceAxes=FollowerAxes  RotationSequence=XYX  RotationSequenceAngles=[0 0 0]  RotationSequenceAnglesUnits=deg  RotationMatrix=[1 0 0; 0 1 0; 0 0 1]
  Transform74 : sm_lib/Frames and Transforms/Rigid Transform  TranslationMethod=Cartesian  TranslationStandardOffset=0  TranslationLengthUnit=mm  TranslationStandardAxis=+Z  TranslationCartesianOffset=smiData.RigidTransform(296).translation  TranslationROffset=0  TranslationROffsetUnits=m  TranslationZOffset=0  TranslationZOffsetUnits=m  TranslationThetaOffset=0  TranslationThetaOffsetUnits=deg  RotationMethod=ArbitraryAxis  RotationAngleUnits=rad  RotationStandardAxis=+Z  RotationAngle=smiData.RigidTransform(296).angle  RotationArbitraryAxis=smiData.RigidTransform(296).axis  FollAlignAxisA=+X  BaseAlignAxisA=+Y  FollAlignAxisB=+Y  BaseAlignAxisB=+Z  RotationSequenceAxes=FollowerAxes  RotationSequence=XYX  RotationSequenceAngles=[0 0 0]  RotationSequenceAnglesUnits=deg  RotationMatrix=[1 0 0; 0 1 0; 0 0 1]
  Transform75 : sm_lib/Frames and Transforms/Rigid Transform  TranslationMethod=Cartesian  TranslationStandardOffset=0  TranslationLengthUnit=mm  TranslationStandardAxis=+Z  TranslationCartesianOffset=smiData.RigidTransform(297).translation  TranslationROffset=0  TranslationROffsetUnits=m  TranslationZOffset=0  TranslationZOffsetUnits=m  TranslationThetaOffset=0  TranslationThetaOffsetUnits=deg  RotationMethod=ArbitraryAxis  RotationAngleUnits=rad  RotationStandardAxis=+Z  RotationAngle=smiData.RigidTransform(297).angle  RotationArbitraryAxis=smiData.RigidTransform(297).axis  FollAlignAxisA=+X  BaseAlignAxisA=+Y  FollAlignAxisB=+Y  BaseAlignAxisB=+Z  RotationSequenceAxes=FollowerAxes  RotationSequence=XYX  RotationSequenceAngles=[0 0 0]  RotationSequenceAnglesUnits=deg  RotationMatrix=[1 0 0; 0 1 0; 0 0 1]
  Transform76 : sm_lib/Frames and Transforms/Rigid Transform  TranslationMethod=Cartesian  TranslationStandardOffset=0  TranslationLengthUnit=mm  TranslationStandardAxis=+Z  TranslationCartesianOffset=smiData.RigidTransform(298).translation  TranslationROffset=0  TranslationROffsetUnits=m  TranslationZOffset=0  TranslationZOffsetUnits=m  TranslationThetaOffset=0  TranslationThetaOffsetUnits=deg  RotationMethod=ArbitraryAxis  RotationAngleUnits=rad  RotationStandardAxis=+Z  RotationAngle=smiData.RigidTransform(298).angle  RotationArbitraryAxis=smiData.RigidTransform(298).axis  FollAlignAxisA=+X  BaseAlignAxisA=+Y  FollAlignAxisB=+Y  BaseAlignAxisB=+Z  RotationSequenceAxes=FollowerAxes  RotationSequence=XYX  RotationSequenceAngles=[0 0 0]  RotationSequenceAnglesUnits=deg  RotationMatrix=[1 0 0; 0 1 0; 0 0 1]
  Transform77 : sm_lib/Frames and Transforms/Rigid Transform  TranslationMethod=Cartesian  TranslationStandardOffset=0  TranslationLengthUnit=mm  TranslationStandardAxis=+Z  TranslationCartesianOffset=smiData.RigidTransform(299).translation  TranslationROffset=0  TranslationROffsetUnits=m  TranslationZOffset=0  TranslationZOffsetUnits=m  TranslationThetaOffset=0  TranslationThetaOffsetUnits=deg  RotationMethod=ArbitraryAxis  RotationAngleUnits=rad  RotationStandardAxis=+Z  RotationAngle=smiData.RigidTransform(299).angle  RotationArbitraryAxis=smiData.RigidTransform(299).axis  FollAlignAxisA=+X  BaseAlignAxisA=+Y  FollAlignAxisB=+Y  BaseAlignAxisB=+Z  RotationSequenceAxes=FollowerAxes  RotationSequence=XYX  RotationSequenceAngles=[0 0 0]  RotationSequenceAnglesUnits=deg  RotationMatrix=[1 0 0; 0 1 0; 0 0 1]
  Transform78 : sm_lib/Frames and Transforms/Rigid Transform  TranslationMethod=Cartesian  TranslationStandardOffset=0  TranslationLengthUnit=mm  TranslationStandardAxis=+Z  TranslationCartesianOffset=smiData.RigidTransform(300).translation  TranslationROffset=0  TranslationROffsetUnits=m  TranslationZOffset=0  TranslationZOffsetUnits=m  TranslationThetaOffset=0  TranslationThetaOffsetUnits=deg  RotationMethod=ArbitraryAxis  RotationAngleUnits=rad  RotationStandardAxis=+Z  RotationAngle=smiData.RigidTransform(300).angle  RotationArbitraryAxis=smiData.RigidTransform(300).axis  FollAlignAxisA=+X  BaseAlignAxisA=+Y  FollAlignAxisB=+Y  BaseAlignAxisB=+Z  RotationSequenceAxes=FollowerAxes  RotationSequence=XYX  RotationSequenceAngles=[0 0 0]  RotationSequenceAnglesUnits=deg  RotationMatrix=[1 0 0; 0 1 0; 0 0 1]
  Transform79 : sm_lib/Frames and Transforms/Rigid Transform  TranslationMethod=Cartesian  TranslationStandardOffset=0  TranslationLengthUnit=mm  TranslationStandardAxis=+Z  TranslationCartesianOffset=smiData.RigidTransform(301).translation  TranslationROffset=0  TranslationROffsetUnits=m  TranslationZOffset=0  TranslationZOffsetUnits=m  TranslationThetaOffset=0  TranslationThetaOffsetUnits=deg  RotationMethod=ArbitraryAxis  RotationAngleUnits=rad  RotationStandardAxis=+Z  RotationAngle=smiData.RigidTransform(301).angle  RotationArbitraryAxis=smiData.RigidTransform(301).axis  FollAlignAxisA=+X  BaseAlignAxisA=+Y  FollAlignAxisB=+Y  BaseAlignAxisB=+Z  RotationSequenceAxes=FollowerAxes  RotationSequence=XYX  RotationSequenceAngles=[0 0 0]  RotationSequenceAnglesUnits=deg  RotationMatrix=[1 0 0; 0 1 0; 0 0 1]
  Transform8 : sm_lib/Frames and Transforms/Rigid Transform  TranslationMethod=Cartesian  TranslationStandardOffset=0  TranslationLengthUnit=mm  TranslationStandardAxis=+Z  TranslationCartesianOffset=smiData.RigidTransform(230).translation  TranslationROffset=0  TranslationROffsetUnits=m  TranslationZOffset=0  TranslationZOffsetUnits=m  TranslationThetaOffset=0  TranslationThetaOffsetUnits=deg  RotationMethod=ArbitraryAxis  RotationAngleUnits=rad  RotationStandardAxis=+Z  RotationAngle=smiData.RigidTransform(230).angle  RotationArbitraryAxis=smiData.RigidTransform(230).axis  FollAlignAxisA=+X  BaseAlignAxisA=+Y  FollAlignAxisB=+Y  BaseAlignAxisB=+Z  RotationSequenceAxes=FollowerAxes  RotationSequence=XYX  RotationSequenceAngles=[0 0 0]  RotationSequenceAnglesUnits=deg  RotationMatrix=[1 0 0; 0 1 0; 0 0 1]
  Transform80 : sm_lib/Frames and Transforms/Rigid Transform  TranslationMethod=Cartesian  TranslationStandardOffset=0  TranslationLengthUnit=mm  TranslationStandardAxis=+Z  TranslationCartesianOffset=smiData.RigidTransform(302).translation  TranslationROffset=0  TranslationROffsetUnits=m  TranslationZOffset=0  TranslationZOffsetUnits=m  TranslationThetaOffset=0  TranslationThetaOffsetUnits=deg  RotationMethod=ArbitraryAxis  RotationAngleUnits=rad  RotationStandardAxis=+Z  RotationAngle=smiData.RigidTransform(302).angle  RotationArbitraryAxis=smiData.RigidTransform(302).axis  FollAlignAxisA=+X  BaseAlignAxisA=+Y  FollAlignAxisB=+Y  BaseAlignAxisB=+Z  RotationSequenceAxes=FollowerAxes  RotationSequence=XYX  RotationSequenceAngles=[0 0 0]  RotationSequenceAnglesUnits=deg  RotationMatrix=[1 0 0; 0 1 0; 0 0 1]
  Transform81 : sm_lib/Frames and Transforms/Rigid Transform  TranslationMethod=Cartesian  TranslationStandardOffset=0  TranslationLengthUnit=mm  TranslationStandardAxis=+Z  TranslationCartesianOffset=smiData.RigidTransform(303).translation  TranslationROffset=0  TranslationROffsetUnits=m  TranslationZOffset=0  TranslationZOffsetUnits=m  TranslationThetaOffset=0  TranslationThetaOffsetUnits=deg  RotationMethod=ArbitraryAxis  RotationAngleUnits=rad  RotationStandardAxis=+Z  RotationAngle=smiData.RigidTransform(303).angle  RotationArbitraryAxis=smiData.RigidTransform(303).axis  FollAlignAxisA=+X  BaseAlignAxisA=+Y  FollAlignAxisB=+Y  BaseAlignAxisB=+Z  RotationSequenceAxes=FollowerAxes  RotationSequence=XYX  RotationSequenceAngles=[0 0 0]  RotationSequenceAnglesUnits=deg  RotationMatrix=[1 0 0; 0 1 0; 0 0 1]
  Transform82 : sm_lib/Frames and Transforms/Rigid Transform  TranslationMethod=Cartesian  TranslationStandardOffset=0  TranslationLengthUnit=mm  TranslationStandardAxis=+Z  TranslationCartesianOffset=smiData.RigidTransform(304).translation  TranslationROffset=0  TranslationROffsetUnits=m  TranslationZOffset=0  TranslationZOffsetUnits=m  TranslationThetaOffset=0  TranslationThetaOffsetUnits=deg  RotationMethod=ArbitraryAxis  RotationAngleUnits=rad  RotationStandardAxis=+Z  RotationAngle=smiData.RigidTransform(304).angle  RotationArbitraryAxis=smiData.RigidTransform(304).axis  FollAlignAxisA=+X  BaseAlignAxisA=+Y  FollAlignAxisB=+Y  BaseAlignAxisB=+Z  RotationSequenceAxes=FollowerAxes  RotationSequence=XYX  RotationSequenceAngles=[0 0 0]  RotationSequenceAnglesUnits=deg  RotationMatrix=[1 0 0; 0 1 0; 0 0 1]
  Transform83 : sm_lib/Frames and Transforms/Rigid Transform  TranslationMethod=Cartesian  TranslationStandardOffset=0  TranslationLengthUnit=mm  TranslationStandardAxis=+Z  TranslationCartesianOffset=smiData.RigidTransform(305).translation  TranslationROffset=0  TranslationROffsetUnits=m  TranslationZOffset=0  TranslationZOffsetUnits=m  TranslationThetaOffset=0  TranslationThetaOffsetUnits=deg  RotationMethod=ArbitraryAxis  RotationAngleUnits=rad  RotationStandardAxis=+Z  RotationAngle=smiData.RigidTransform(305).angle  RotationArbitraryAxis=smiData.RigidTransform(305).axis  FollAlignAxisA=+X  BaseAlignAxisA=+Y  FollAlignAxisB=+Y  BaseAlignAxisB=+Z  RotationSequenceAxes=FollowerAxes  RotationSequence=XYX  RotationSequenceAngles=[0 0 0]  RotationSequenceAnglesUnits=deg  RotationMatrix=[1 0 0; 0 1 0; 0 0 1]
  Transform84 : sm_lib/Frames and Transforms/Rigid Transform  TranslationMethod=Cartesian  TranslationStandardOffset=0  TranslationLengthUnit=mm  TranslationStandardAxis=+Z  TranslationCartesianOffset=smiData.RigidTransform(306).translation  TranslationROffset=0  TranslationROffsetUnits=m  TranslationZOffset=0  TranslationZOffsetUnits=m  TranslationThetaOffset=0  TranslationThetaOffsetUnits=deg  RotationMethod=ArbitraryAxis  RotationAngleUnits=rad  RotationStandardAxis=+Z  RotationAngle=smiData.RigidTransform(306).angle  RotationArbitraryAxis=smiData.RigidTransform(306).axis  FollAlignAxisA=+X  BaseAlignAxisA=+Y  FollAlignAxisB=+Y  BaseAlignAxisB=+Z  RotationSequenceAxes=FollowerAxes  RotationSequence=XYX  RotationSequenceAngles=[0 0 0]  RotationSequenceAnglesUnits=deg  RotationMatrix=[1 0 0; 0 1 0; 0 0 1]
  Transform85 : sm_lib/Frames and Transforms/Rigid Transform  TranslationMethod=Cartesian  TranslationStandardOffset=0  TranslationLengthUnit=mm  TranslationStandardAxis=+Z  TranslationCartesianOffset=smiData.RigidTransform(307).translation  TranslationROffset=0  TranslationROffsetUnits=m  TranslationZOffset=0  TranslationZOffsetUnits=m  TranslationThetaOffset=0  TranslationThetaOffsetUnits=deg  RotationMethod=ArbitraryAxis  RotationAngleUnits=rad  RotationStandardAxis=+Z  RotationAngle=smiData.RigidTransform(307).angle  RotationArbitraryAxis=smiData.RigidTransform(307).axis  FollAlignAxisA=+X  BaseAlignAxisA=+Y  FollAlignAxisB=+Y  BaseAlignAxisB=+Z  RotationSequenceAxes=FollowerAxes  RotationSequence=XYX  RotationSequenceAngles=[0 0 0]  RotationSequenceAnglesUnits=deg  RotationMatrix=[1 0 0; 0 1 0; 0 0 1]
  Transform86 : sm_lib/Frames and Transforms/Rigid Transform  TranslationMethod=Cartesian  TranslationStandardOffset=0  TranslationLengthUnit=mm  TranslationStandardAxis=+Z  TranslationCartesianOffset=smiData.RigidTransform(308).translation  TranslationROffset=0  TranslationROffsetUnits=m  TranslationZOffset=0  TranslationZOffsetUnits=m  TranslationThetaOffset=0  TranslationThetaOffsetUnits=deg  RotationMethod=ArbitraryAxis  RotationAngleUnits=rad  RotationStandardAxis=+Z  RotationAngle=smiData.RigidTransform(308).angle  RotationArbitraryAxis=smiData.RigidTransform(308).axis  FollAlignAxisA=+X  BaseAlignAxisA=+Y  FollAlignAxisB=+Y  BaseAlignAxisB=+Z  RotationSequenceAxes=FollowerAxes  RotationSequence=XYX  RotationSequenceAngles=[0 0 0]  RotationSequenceAnglesUnits=deg  RotationMatrix=[1 0 0; 0 1 0; 0 0 1]
  Transform87 : sm_lib/Frames and Transforms/Rigid Transform  TranslationMethod=Cartesian  TranslationStandardOffset=0  TranslationLengthUnit=mm  TranslationStandardAxis=+Z  TranslationCartesianOffset=smiData.RigidTransform(309).translation  TranslationROffset=0  TranslationROffsetUnits=m  TranslationZOffset=0  TranslationZOffsetUnits=m  TranslationThetaOffset=0  TranslationThetaOffsetUnits=deg  RotationMethod=ArbitraryAxis  RotationAngleUnits=rad  RotationStandardAxis=+Z  RotationAngle=smiData.RigidTransform(309).angle  RotationArbitraryAxis=smiData.RigidTransform(309).axis  FollAlignAxisA=+X  BaseAlignAxisA=+Y  FollAlignAxisB=+Y  BaseAlignAxisB=+Z  RotationSequenceAxes=FollowerAxes  RotationSequence=XYX  RotationSequenceAngles=[0 0 0]  RotationSequenceAnglesUnits=deg  RotationMatrix=[1 0 0; 0 1 0; 0 0 1]
  Transform88 : sm_lib/Frames and Transforms/Rigid Transform  TranslationMethod=Cartesian  TranslationStandardOffset=0  TranslationLengthUnit=mm  TranslationStandardAxis=+Z  TranslationCartesianOffset=smiData.RigidTransform(310).translation  TranslationROffset=0  TranslationROffsetUnits=m  TranslationZOffset=0  TranslationZOffsetUnits=m  TranslationThetaOffset=0  TranslationThetaOffsetUnits=deg  RotationMethod=ArbitraryAxis  RotationAngleUnits=rad  RotationStandardAxis=+Z  RotationAngle=smiData.RigidTransform(310).angle  RotationArbitraryAxis=smiData.RigidTransform(310).axis  FollAlignAxisA=+X  BaseAlignAxisA=+Y  FollAlignAxisB=+Y  BaseAlignAxisB=+Z  RotationSequenceAxes=FollowerAxes  RotationSequence=XYX  RotationSequenceAngles=[0 0 0]  RotationSequenceAnglesUnits=deg  RotationMatrix=[1 0 0; 0 1 0; 0 0 1]
  Transform89 : sm_lib/Frames and Transforms/Rigid Transform  TranslationMethod=Cartesian  TranslationStandardOffset=0  TranslationLengthUnit=mm  TranslationStandardAxis=+Z  TranslationCartesianOffset=smiData.RigidTransform(311).translation  TranslationROffset=0  TranslationROffsetUnits=m  TranslationZOffset=0  TranslationZOffsetUnits=m  TranslationThetaOffset=0  TranslationThetaOffsetUnits=deg  RotationMethod=ArbitraryAxis  RotationAngleUnits=rad  RotationStandardAxis=+Z  RotationAngle=smiData.RigidTransform(311).angle  RotationArbitraryAxis=smiData.RigidTransform(311).axis  FollAlignAxisA=+X  BaseAlignAxisA=+Y  FollAlignAxisB=+Y  BaseAlignAxisB=+Z  RotationSequenceAxes=FollowerAxes  RotationSequence=XYX  RotationSequenceAngles=[0 0 0]  RotationSequenceAnglesUnits=deg  RotationMatrix=[1 0 0; 0 1 0; 0 0 1]
  Transform9 : sm_lib/Frames and Transforms/Rigid Transform  TranslationMethod=Cartesian  TranslationStandardOffset=0  TranslationLengthUnit=mm  TranslationStandardAxis=+Z  TranslationCartesianOffset=smiData.RigidTransform(231).translation  TranslationROffset=0  TranslationROffsetUnits=m  TranslationZOffset=0  TranslationZOffsetUnits=m  TranslationThetaOffset=0  TranslationThetaOffsetUnits=deg  RotationMethod=ArbitraryAxis  RotationAngleUnits=rad  RotationStandardAxis=+Z  RotationAngle=smiData.RigidTransform(231).angle  RotationArbitraryAxis=smiData.RigidTransform(231).axis  FollAlignAxisA=+X  BaseAlignAxisA=+Y  FollAlignAxisB=+Y  BaseAlignAxisB=+Z  RotationSequenceAxes=FollowerAxes  RotationSequence=XYX  RotationSequenceAngles=[0 0 0]  RotationSequenceAnglesUnits=deg  RotationMatrix=[1 0 0; 0 1 0; 0 0 1]
  Transform90 : sm_lib/Frames and Transforms/Rigid Transform  TranslationMethod=Cartesian  TranslationStandardOffset=0  TranslationLengthUnit=mm  TranslationStandardAxis=+Z  TranslationCartesianOffset=smiData.RigidTransform(312).translation  TranslationROffset=0  TranslationROffsetUnits=m  TranslationZOffset=0  TranslationZOffsetUnits=m  TranslationThetaOffset=0  TranslationThetaOffsetUnits=deg  RotationMethod=ArbitraryAxis  RotationAngleUnits=rad  RotationStandardAxis=+Z  RotationAngle=smiData.RigidTransform(312).angle  RotationArbitraryAxis=smiData.RigidTransform(312).axis  FollAlignAxisA=+X  BaseAlignAxisA=+Y  FollAlignAxisB=+Y  BaseAlignAxisB=+Z  RotationSequenceAxes=FollowerAxes  RotationSequence=XYX  RotationSequenceAngles=[0 0 0]  RotationSequenceAnglesUnits=deg  RotationMatrix=[1 0 0; 0 1 0; 0 0 1]
  Transform91 : sm_lib/Frames and Transforms/Rigid Transform  TranslationMethod=Cartesian  TranslationStandardOffset=0  TranslationLengthUnit=mm  TranslationStandardAxis=+Z  TranslationCartesianOffset=smiData.RigidTransform(313).translation  TranslationROffset=0  TranslationROffsetUnits=m  TranslationZOffset=0  TranslationZOffsetUnits=m  TranslationThetaOffset=0  TranslationThetaOffsetUnits=deg  RotationMethod=ArbitraryAxis  RotationAngleUnits=rad  RotationStandardAxis=+Z  RotationAngle=smiData.RigidTransform(313).angle  RotationArbitraryAxis=smiData.RigidTransform(313).axis  FollAlignAxisA=+X  BaseAlignAxisA=+Y  FollAlignAxisB=+Y  BaseAlignAxisB=+Z  RotationSequenceAxes=FollowerAxes  RotationSequence=XYX  RotationSequenceAngles=[0 0 0]  RotationSequenceAnglesUnits=deg  RotationMatrix=[1 0 0; 0 1 0; 0 0 1]
  Transform92 : sm_lib/Frames and Transforms/Rigid Transform  TranslationMethod=Cartesian  TranslationStandardOffset=0  TranslationLengthUnit=mm  TranslationStandardAxis=+Z  TranslationCartesianOffset=smiData.RigidTransform(314).translation  TranslationROffset=0  TranslationROffsetUnits=m  TranslationZOffset=0  TranslationZOffsetUnits=m  TranslationThetaOffset=0  TranslationThetaOffsetUnits=deg  RotationMethod=ArbitraryAxis  RotationAngleUnits=rad  RotationStandardAxis=+Z  RotationAngle=smiData.RigidTransform(314).angle  RotationArbitraryAxis=smiData.RigidTransform(314).axis  FollAlignAxisA=+X  BaseAlignAxisA=+Y  FollAlignAxisB=+Y  BaseAlignAxisB=+Z  RotationSequenceAxes=FollowerAxes  RotationSequence=XYX  RotationSequenceAngles=[0 0 0]  RotationSequenceAnglesUnits=deg  RotationMatrix=[1 0 0; 0 1 0; 0 0 1]
  Transform93 : sm_lib/Frames and Transforms/Rigid Transform  TranslationMethod=Cartesian  TranslationStandardOffset=0  TranslationLengthUnit=mm  TranslationStandardAxis=+Z  TranslationCartesianOffset=smiData.RigidTransform(315).translation  TranslationROffset=0  TranslationROffsetUnits=m  TranslationZOffset=0  TranslationZOffsetUnits=m  TranslationThetaOffset=0  TranslationThetaOffsetUnits=deg  RotationMethod=ArbitraryAxis  RotationAngleUnits=rad  RotationStandardAxis=+Z  RotationAngle=smiData.RigidTransform(315).angle  RotationArbitraryAxis=smiData.RigidTransform(315).axis  FollAlignAxisA=+X  BaseAlignAxisA=+Y  FollAlignAxisB=+Y  BaseAlignAxisB=+Z  RotationSequenceAxes=FollowerAxes  RotationSequence=XYX  RotationSequenceAngles=[0 0 0]  RotationSequenceAnglesUnits=deg  RotationMatrix=[1 0 0; 0 1 0; 0 0 1]
  Transform94 : sm_lib/Frames and Transforms/Rigid Transform  TranslationMethod=Cartesian  TranslationStandardOffset=0  TranslationLengthUnit=mm  TranslationStandardAxis=+Z  TranslationCartesianOffset=smiData.RigidTransform(316).translation  TranslationROffset=0  TranslationROffsetUnits=m  TranslationZOffset=0  TranslationZOffsetUnits=m  TranslationThetaOffset=0  TranslationThetaOffsetUnits=deg  RotationMethod=ArbitraryAxis  RotationAngleUnits=rad  RotationStandardAxis=+Z  RotationAngle=smiData.RigidTransform(316).angle  RotationArbitraryAxis=smiData.RigidTransform(316).axis  FollAlignAxisA=+X  BaseAlignAxisA=+Y  FollAlignAxisB=+Y  BaseAlignAxisB=+Z  RotationSequenceAxes=FollowerAxes  RotationSequence=XYX  RotationSequenceAngles=[0 0 0]  RotationSequenceAnglesUnits=deg  RotationMatrix=[1 0 0; 0 1 0; 0 0 1]
  Transform95 : sm_lib/Frames and Transforms/Rigid Transform  TranslationMethod=Cartesian  TranslationStandardOffset=0  TranslationLengthUnit=mm  TranslationStandardAxis=+Z  TranslationCartesianOffset=smiData.RigidTransform(317).translation  TranslationROffset=0  TranslationROffsetUnits=m  TranslationZOffset=0  TranslationZOffsetUnits=m  TranslationThetaOffset=0  TranslationThetaOffsetUnits=deg  RotationMethod=ArbitraryAxis  RotationAngleUnits=rad  RotationStandardAxis=+Z  RotationAngle=smiData.RigidTransform(317).angle  RotationArbitraryAxis=smiData.RigidTransform(317).axis  FollAlignAxisA=+X  BaseAlignAxisA=+Y  FollAlignAxisB=+Y  BaseAlignAxisB=+Z  RotationSequenceAxes=FollowerAxes  RotationSequence=XYX  RotationSequenceAngles=[0 0 0]  RotationSequenceAnglesUnits=deg  RotationMatrix=[1 0 0; 0 1 0; 0 0 1]
  Transform96 : sm_lib/Frames and Transforms/Rigid Transform  TranslationMethod=Cartesian  TranslationStandardOffset=0  TranslationLengthUnit=mm  TranslationStandardAxis=+Z  TranslationCartesianOffset=smiData.RigidTransform(318).translation  TranslationROffset=0  TranslationROffsetUnits=m  TranslationZOffset=0  TranslationZOffsetUnits=m  TranslationThetaOffset=0  TranslationThetaOffsetUnits=deg  RotationMethod=ArbitraryAxis  RotationAngleUnits=rad  RotationStandardAxis=+Z  RotationAngle=smiData.RigidTransform(318).angle  RotationArbitraryAxis=smiData.RigidTransform(318).axis  FollAlignAxisA=+X  BaseAlignAxisA=+Y  FollAlignAxisB=+Y  BaseAlignAxisB=+Z  RotationSequenceAxes=FollowerAxes  RotationSequence=XYX  RotationSequenceAngles=[0 0 0]  RotationSequenceAnglesUnits=deg  RotationMatrix=[1 0 0; 0 1 0; 0 0 1]
  Transform97 : sm_lib/Frames and Transforms/Rigid Transform  TranslationMethod=Cartesian  TranslationStandardOffset=0  TranslationLengthUnit=mm  TranslationStandardAxis=+Z  TranslationCartesianOffset=smiData.RigidTransform(319).translation  TranslationROffset=0  TranslationROffsetUnits=m  TranslationZOffset=0  TranslationZOffsetUnits=m  TranslationThetaOffset=0  TranslationThetaOffsetUnits=deg  RotationMethod=ArbitraryAxis  RotationAngleUnits=rad  RotationStandardAxis=+Z  RotationAngle=smiData.RigidTransform(319).angle  RotationArbitraryAxis=smiData.RigidTransform(319).axis  FollAlignAxisA=+X  BaseAlignAxisA=+Y  FollAlignAxisB=+Y  BaseAlignAxisB=+Z  RotationSequenceAxes=FollowerAxes  RotationSequence=XYX  RotationSequenceAngles=[0 0 0]  RotationSequenceAnglesUnits=deg  RotationMatrix=[1 0 0; 0 1 0; 0 0 1]
  Transform98 : sm_lib/Frames and Transforms/Rigid Transform  TranslationMethod=Cartesian  TranslationStandardOffset=0  TranslationLengthUnit=mm  TranslationStandardAxis=+Z  TranslationCartesianOffset=smiData.RigidTransform(320).translation  TranslationROffset=0  TranslationROffsetUnits=m  TranslationZOffset=0  TranslationZOffsetUnits=m  TranslationThetaOffset=0  TranslationThetaOffsetUnits=deg  RotationMethod=ArbitraryAxis  RotationAngleUnits=rad  RotationStandardAxis=+Z  RotationAngle=smiData.RigidTransform(320).angle  RotationArbitraryAxis=smiData.RigidTransform(320).axis  FollAlignAxisA=+X  BaseAlignAxisA=+Y  FollAlignAxisB=+Y  BaseAlignAxisB=+Z  RotationSequenceAxes=FollowerAxes  RotationSequence=XYX  RotationSequenceAngles=[0 0 0]  RotationSequenceAnglesUnits=deg  RotationMatrix=[1 0 0; 0 1 0; 0 0 1]
  Transform99 : sm_lib/Frames and Transforms/Rigid Transform  TranslationMethod=Cartesian  TranslationStandardOffset=0  TranslationLengthUnit=mm  TranslationStandardAxis=+Z  TranslationCartesianOffset=smiData.RigidTransform(321).translation  TranslationROffset=0  TranslationROffsetUnits=m  TranslationZOffset=0  TranslationZOffsetUnits=m  TranslationThetaOffset=0  TranslationThetaOffsetUnits=deg  RotationMethod=ArbitraryAxis  RotationAngleUnits=rad  RotationStandardAxis=+Z  RotationAngle=smiData.RigidTransform(321).angle  RotationArbitraryAxis=smiData.RigidTransform(321).axis  FollAlignAxisA=+X  BaseAlignAxisA=+Y  FollAlignAxisB=+Y  BaseAlignAxisB=+Z  RotationSequenceAxes=FollowerAxes  RotationSequence=XYX  RotationSequenceAngles=[0 0 0]  RotationSequenceAnglesUnits=deg  RotationMatrix=[1 0 0; 0 1 0; 0 0 1]
  User_Library_15x28x7_brg_1_RIGID : Subsystem
  User_Library_15x28x7_brg_2_RIGID : Subsystem
  formed_hex_screw_am_10_RIGID : Subsystem
  formed_hex_screw_am_11_RIGID : Subsystem
  formed_hex_screw_am_12_RIGID : Subsystem
  formed_hex_screw_am_13_RIGID : Subsystem
  formed_hex_screw_am_15_RIGID : Subsystem
  formed_hex_screw_am_16_RIGID : Subsystem
  formed_hex_screw_am_17_RIGID : Subsystem
  formed_hex_screw_am_18_RIGID : Subsystem
  formed_hex_screw_am_19_RIGID : Subsystem
  formed_hex_screw_am_1_RIGID : Subsystem
  formed_hex_screw_am_20_RIGID : Subsystem
  formed_hex_screw_am_22_RIGID : Subsystem
  formed_hex_screw_am_24_RIGID : Subsystem
  formed_hex_screw_am_4_RIGID : Subsystem
  formed_hex_screw_am_5_RIGID : Subsystem
  formed_hex_screw_am_6_RIGID : Subsystem
  formed_hex_screw_am_9_RIGID : Subsystem
  hex_nut_jam_am_3_RIGID : Subsystem
  hex_nut_style_1_am_11_RIGID : Subsystem
  hex_nut_style_1_am_12_RIGID : Subsystem
  hex_nut_style_1_am_13_RIGID : Subsystem
  hex_nut_style_1_am_14_RIGID : Subsystem
  hex_nut_style_1_am_2_RIGID : Subsystem
  hex_nut_style_1_am_3_RIGID : Subsystem
  hex_nut_style_1_am_4_RIGID : Subsystem
  hex_nut_style_1_am_5_RIGID : Subsystem
  hex_nut_style_1_am_6_RIGID : Subsystem
  hex_nut_style_1_am_7_RIGID : Subsystem
  hex_nut_style_1_am_8_RIGID : Subsystem
  hex_nut_style_1_am_9_RIGID : Subsystem
  hex_nut_style_2_ams_2_RIGID : Subsystem
  hex_screw_am_10_RIGID : Subsystem
  hex_screw_am_11_RIGID : Subsystem
  hex_screw_am_12_RIGID : Subsystem
  hex_screw_am_13_RIGID : Subsystem
  hex_screw_am_14_RIGID : Subsystem
  hex_screw_am_15_RIGID : Subsystem
  hex_screw_am_16_RIGID : Subsystem
  hex_screw_am_17_RIGID : Subsystem
  hex_screw_am_18_RIGID : Subsystem
  hex_screw_am_19_RIGID : Subsystem
  hex_screw_am_1_RIGID : Subsystem
  hex_screw_am_20_RIGID : Subsystem
  hex_screw_am_22_RIGID : Subsystem
  hex_screw_am_23_RIGID : Subsystem
  hex_screw_am_24_RIGID : Subsystem
  hex_screw_am_25_RIGID : Subsystem
  hex_screw_am_26_RIGID : Subsystem
  hex_screw_am_27_RIGID : Subsystem
  hex_screw_am_28_RIGID : Subsystem
  hex_screw_am_29_RIGID : Subsystem
  hex_screw_am_2_RIGID : Subsystem
  hex_screw_am_3_RIGID : Subsystem
  hex_screw_am_5_RIGID : Subsystem
  hex_screw_am_6_RIGID : Subsystem
  hex_screw_am_7_RIGID : Subsystem
  hex_screw_am_8_RIGID : Subsystem
  hex_screw_am_9_RIGID : Subsystem
  instrument_ball_bearing_68_am_100_RIGID : Subsystem
  instrument_ball_bearing_68_am_101_RIGID : Subsystem
  instrument_ball_bearing_68_am_102_RIGID : Subsystem
  instrument_ball_bearing_68_am_103_RIGID : Subsystem
  instrument_ball_bearing_68_am_104_RIGID : Subsystem
  instrument_ball_bearing_68_am_105_RIGID : Subsystem
  instrument_ball_bearing_68_am_11_RIGID : Subsystem
  instrument_ball_bearing_68_am_12_RIGID : Subsystem
  instrument_ball_bearing_68_am_13_RIGID : Subsystem
  instrument_ball_bearing_68_am_14_RIGID : Subsystem
  instrument_ball_bearing_68_am_15_RIGID : Subsystem
  instrument_ball_bearing_68_am_16_RIGID : Subsystem
  instrument_ball_bearing_68_am_17_RIGID : Subsystem
  instrument_ball_bearing_68_am_18_RIGID : Subsystem
  instrument_ball_bearing_68_am_19_RIGID : Subsystem
  instrument_ball_bearing_68_am_20_RIGID : Subsystem
  instrument_ball_bearing_68_am_21_RIGID : Subsystem
  instrument_ball_bearing_68_am_22_RIGID : Subsystem
  instrument_ball_bearing_68_am_23_RIGID : Subsystem
  instrument_ball_bearing_68_am_24_RIGID : Subsystem
  instrument_ball_bearing_68_am_25_RIGID : Subsystem
  instrument_ball_bearing_68_am_26_RIGID : Subsystem
  instrument_ball_bearing_68_am_27_RIGID : Subsystem
  instrument_ball_bearing_68_am_28_RIGID : Subsystem
  instrument_ball_bearing_68_am_29_RIGID : Subsystem
  instrument_ball_bearing_68_am_30_RIGID : Subsystem
  instrument_ball_bearing_68_am_31_RIGID : Subsystem
  instrument_ball_bearing_68_am_32_RIGID : Subsystem
  instrument_ball_bearing_68_am_33_RIGID : Subsystem
  instrument_ball_bearing_68_am_34_RIGID : Subsystem
  instrument_ball_bearing_68_am_35_RIGID : Subsystem
  instrument_ball_bearing_68_am_36_RIGID : Subsystem
  instrument_ball_bearing_68_am_37_RIGID : Subsystem
  instrument_ball_bearing_68_am_38_RIGID : Subsystem
  instrument_ball_bearing_68_am_39_RIGID : Subsystem
  instrument_ball_bearing_68_am_40_RIGID : Subsystem
  instrument_ball_bearing_68_am_41_RIGID : Subsystem
  instrument_ball_bearing_68_am_42_RIGID : Subsystem
  instrument_ball_bearing_68_am_43_RIGID : Subsystem
  instrument_ball_bearing_68_am_44_RIGID : Subsystem
  instrument_ball_bearing_68_am_45_RIGID : Subsystem
  instrument_ball_bearing_68_am_46_RIGID : Subsystem
  instrument_ball_bearing_68_am_47_RIGID : Subsystem
  instrument_ball_bearing_68_am_48_RIGID : Subsystem
  instrument_ball_bearing_68_am_49_RIGID : Subsystem
  instrument_ball_bearing_68_am_4_RIGID : Subsystem
  instrument_ball_bearing_68_am_52_RIGID : Subsystem
  instrument_ball_bearing_68_am_53_RIGID : Subsystem
  instrument_ball_bearing_68_am_54_RIGID : Subsystem
  instrument_ball_bearing_68_am_55_RIGID : Subsystem
  instrument_ball_bearing_68_am_56_RIGID : Subsystem
  instrument_ball_bearing_68_am_57_RIGID : Subsystem
  instrument_ball_bearing_68_am_58_RIGID : Subsystem
  instrument_ball_bearing_68_am_59_RIGID : Subsystem
  instrument_ball_bearing_68_am_5_RIGID : Subsystem
  instrument_ball_bearing_68_am_60_RIGID : Subsystem
  instrument_ball_bearing_68_am_61_RIGID : Subsystem
  instrument_ball_bearing_68_am_62_RIGID : Subsystem
  instrument_ball_bearing_68_am_63_RIGID : Subsystem
  instrument_ball_bearing_68_am_64_RIGID : Subsystem
  instrument_ball_bearing_68_am_65_RIGID : Subsystem
  instrument_ball_bearing_68_am_66_RIGID : Subsystem
  instrument_ball_bearing_68_am_67_RIGID : Subsystem
  instrument_ball_bearing_68_am_68_RIGID : Subsystem
  instrument_ball_bearing_68_am_69_RIGID : Subsystem
  instrument_ball_bearing_68_am_6_RIGID : Subsystem
  instrument_ball_bearing_68_am_70_RIGID : Subsystem
  instrument_ball_bearing_68_am_71_RIGID : Subsystem
  instrument_ball_bearing_68_am_72_RIGID : Subsystem
  instrument_ball_bearing_68_am_73_RIGID : Subsystem
  instrument_ball_bearing_68_am_74_RIGID : Subsystem
  instrument_ball_bearing_68_am_75_RIGID : Subsystem
  instrument_ball_bearing_68_am_76_RIGID : Subsystem
  instrument_ball_bearing_68_am_77_RIGID : Subsystem
  instrument_ball_bearing_68_am_78_RIGID : Subsystem
  instrument_ball_bearing_68_am_79_RIGID : Subsystem
  instrument_ball_bearing_68_am_80_RIGID : Subsystem
  instrument_ball_bearing_68_am_81_RIGID : Subsystem
  instrument_ball_bearing_68_am_82_RIGID : Subsystem
  instrument_ball_bearing_68_am_83_RIGID : Subsystem
  instrument_ball_bearing_68_am_84_RIGID : Subsystem
  instrument_ball_bearing_68_am_85_RIGID : Subsystem
  instrument_ball_bearing_68_am_86_RIGID : Subsystem
  instrument_ball_bearing_68_am_87_RIGID : Subsystem
  instrument_ball_bearing_68_am_88_RIGID : Subsystem
  instrument_ball_bearing_68_am_89_RIGID : Subsystem
  instrument_ball_bearing_68_am_90_RIGID : Subsystem
  instrument_ball_bearing_68_am_91_RIGID : Subsystem
  instrument_ball_bearing_68_am_92_RIGID : Subsystem
  instrument_ball_bearing_68_am_93_RIGID : Subsystem
  instrument_ball_bearing_68_am_94_RIGID : Subsystem
  instrument_ball_bearing_68_am_95_RIGID : Subsystem
  instrument_ball_bearing_68_am_96_RIGID : Subsystem
  instrument_ball_bearing_68_am_97_RIGID : Subsystem
  instrument_ball_bearing_68_am_98_RIGID : Subsystem
  instrument_ball_bearing_68_am_99_RIGID : Subsystem
  pan_cross_head_am_44_RIGID : Subsystem
  pan_cross_head_am_45_RIGID : Subsystem
  pan_cross_head_am_46_RIGID : Subsystem
  pan_cross_head_am_47_RIGID : Subsystem
  pan_cross_head_am_48_RIGID : Subsystem
  pan_cross_head_am_49_RIGID : Subsystem
  pan_cross_head_am_50_RIGID : Subsystem
  pan_cross_head_am_51_RIGID : Subsystem
  pan_cross_head_am_52_RIGID : Subsystem
  pan_cross_head_am_53_RIGID : Subsystem
  pan_cross_head_am_54_RIGID : Subsystem
  pan_cross_head_am_55_RIGID : Subsystem
  pan_cross_head_am_56_RIGID : Subsystem
  pan_cross_head_am_57_RIGID : Subsystem
  pan_cross_head_am_58_RIGID : Subsystem
  pan_cross_head_am_59_RIGID : Subsystem
  pan_cross_head_am_60_RIGID : Subsystem
  pan_cross_head_am_61_RIGID : Subsystem
  pan_cross_head_am_62_RIGID : Subsystem
  pan_cross_head_am_63_RIGID : Subsystem
  pan_cross_head_am_64_RIGID : Subsystem
  pan_cross_head_am_65_RIGID : Subsystem
  pan_cross_head_am_66_RIGID : Subsystem
  pan_cross_head_am_67_RIGID : Subsystem
  pan_cross_head_am_68_RIGID : Subsystem
  pan_cross_head_am_69_RIGID : Subsystem
  pan_cross_head_am_70_RIGID : Subsystem
  pan_cross_head_am_71_RIGID : Subsystem
  pan_cross_head_am_72_RIGID : Subsystem
  pan_cross_head_am_73_RIGID : Subsystem
  pan_cross_head_am_74_RIGID : Subsystem
  pan_cross_head_am_75_RIGID : Subsystem
  pan_cross_head_am_76_RIGID : Subsystem
  pan_cross_head_am_77_RIGID : Subsystem
  pan_cross_head_am_78_RIGID : Subsystem
  socket_set_screw_cone_point_am_1_RIGID : Subsystem
  x15_1_CycloDisk_1_RIGID : Subsystem
  x15_1_CycloDisk_2_RIGID : Subsystem
  x36_Teeth_Pulley_1_RIGID : Subsystem
  F1 : PMIOPort  Side=Left
  F : PMIOPort  Port=2  Side=Right
  connections:
  Transform/LConn1 -- ReferenceFrame/RConn1 -- Transform1/LConn1 -- Transform10/LConn1 -- Transform100/LConn1 -- Transform101/LConn1 -- Transform102/LConn1 -- Transform103/LConn1 -- Transform104/LConn1 -- Transform105/LConn1 -- Transform106/LConn1 -- Transform107/LConn1 -- Transform108/LConn1 -- Transform109/LConn1 -- Transform11/LConn1 -- Transform110/LConn1 -- Transform111/LConn1 -- Transform112/LConn1 -- Transform113/LConn1 -- Transform114/LConn1 -- Transform115/LConn1 -- Transform116/LConn1 -- Transform117/LConn1 -- Transform118/LConn1 -- Transform119/LConn1 -- Transform12/LConn1 -- Transform120/LConn1 -- Transform121/LConn1 -- Transform122/LConn1 -- Transform123/LConn1 -- Transform124/LConn1 -- Transform125/LConn1 -- Transform126/LConn1 -- Transform127/LConn1 -- Transform128/LConn1 -- Transform129/LConn1 -- Transform13/LConn1 -- Transform130/LConn1 -- Transform131/LConn1 -- Transform132/LConn1 -- Transform133/LConn1 -- Transform134/LConn1 -- Transform135/LConn1 -- Transform136/LConn1 -- Transform137/LConn1 -- Transform138/LConn1 -- Transform139/LConn1 -- Transform14/LConn1 -- Transform140/LConn1 -- Transform141/LConn1 -- Transform142/LConn1 -- Transform143/LConn1 -- Transform144/LConn1 -- Transform145/LConn1 -- Transform146/LConn1 -- Transform147/LConn1 -- Transform148/LConn1 -- Transform149/LConn1 -- Transform15/LConn1 -- Transform150/LConn1 -- Transform151/LConn1 -- Transform152/LConn1 -- Transform153/LConn1 -- Transform154/LConn1 -- Transform155/LConn1 -- Transform156/LConn1 -- Transform157/LConn1 -- Transform158/LConn1 -- Transform159/LConn1 -- Transform16/LConn1 -- Transform160/LConn1 -- Transform161/LConn1 -- Transform162/LConn1 -- Transform163/LConn1 -- Transform164/LConn1 -- Transform165/LConn1 -- Transform166/LConn1 -- Transform167/LConn1 -- Transform168/LConn1 -- Transform169/LConn1 -- Transform17/LConn1 -- Transform170/LConn1 -- Transform171/LConn1 -- Transform172/LConn1 -- Transform173/LConn1 -- Transform174/LConn1 -- Transform175/LConn1 -- Transform176/LConn1 -- Transform177/LConn1 -- Transform178/LConn1 -- Transform179/LConn1 -- Transform18/LConn1 -- Transform180/LConn1 -- Transform181/LConn1 -- Transform182/LConn1 -- Transform183/LConn1 -- Transform184/LConn1 -- Transform185/LConn1 -- Transform186/LConn1 -- Transform187/LConn1 -- Transform188/LConn1 -- Transform189/LConn1 -- Transform19/LConn1 -- Transform190/LConn1 -- Transform191/LConn1 -- Transform192/LConn1 -- Transform193/LConn1 -- Transform194/LConn1 -- Transform195/LConn1 -- Transform196/LConn1 -- Transform197/LConn1 -- Transform198/LConn1 -- Transform199/LConn1 -- Transform2/LConn1 -- Transform20/LConn1 -- Transform200/LConn1 -- Transform201/LConn1 -- Transform202/LConn1 -- Transform203/LConn1 -- Transform204/LConn1 -- Transform205/LConn1 -- Transform206/LConn1 -- Transform207/LConn1 -- Transform208/LConn1 -- Transform209/LConn1 -- Transform21/LConn1 -- Transform210/LConn1 -- Transform211/LConn1 -- Transform212/LConn1 -- Transform213/LConn1 -- Transform214/LConn1 -- Transform215/LConn1 -- Transform216/LConn1 -- Transform217/LConn1 -- Transform218/LConn1 -- Transform219/LConn1 -- Transform22/LConn1 -- Transform220/LConn1 -- Transform221/LConn1 -- Transform222/LConn1 -- Transform223/LConn1 -- Transform224/LConn1 -- Transform225/LConn1 -- Transform226/LConn1 -- Transform227/LConn1 -- Transform228/LConn1 -- Transform229/LConn1 -- Transform23/LConn1 -- Transform230/LConn1 -- Transform231/LConn1 -- Transform232/LConn1 -- Transform233/LConn1 -- Transform234/LConn1 -- Transform235/LConn1 -- Transform236/LConn1 -- Transform24/LConn1 -- Transform25/LConn1 -- Transform26/LConn1 -- Transform27/LConn1 -- Transform28/LConn1 -- Transform29/LConn1 -- Transform3/LConn1 -- Transform30/LConn1 -- Transform31/LConn1 -- Transform32/LConn1 -- Transform33/LConn1 -- Transform34/LConn1 -- Transform35/LConn1 -- Transform36/LConn1 -- Transform37/LConn1 -- Transform38/LConn1 -- Transform39/LConn1 -- Transform4/LConn1 -- Transform40/LConn1 -- Transform41/LConn1 -- Transform42/LConn1 -- Transform43/LConn1 -- Transform44/LConn1 -- Transform45/LConn1 -- Transform46/LConn1 -- Transform47/LConn1 -- Transform48/LConn1 -- Transform49/LConn1 -- Transform5/LConn1 -- Transform50/LConn1 -- Transform51/LConn1 -- Transform52/LConn1 -- Transform53/LConn1 -- Transform54/LConn1 -- Transform55/LConn1 -- Transform56/LConn1 -- Transform57/LConn1 -- Transform58/LConn1 -- Transform59/LConn1 -- Transform6/LConn1 -- Transform60/LConn1 -- Transform61/LConn1 -- Transform62/LConn1 -- Transform63/LConn1 -- Transform64/LConn1 -- Transform65/LConn1 -- Transform66/LConn1 -- Transform67/LConn1 -- Transform68/LConn1 -- Transform69/LConn1 -- Transform7/LConn1 -- Transform70/LConn1 -- Transform71/LConn1 -- Transform72/LConn1 -- Transform73/LConn1 -- Transform74/LConn1 -- Transform75/LConn1 -- Transform76/LConn1 -- Transform77/LConn1 -- Transform78/LConn1 -- Transform79/LConn1 -- Transform8/LConn1 -- Transform80/LConn1 -- Transform81/LConn1 -- Transform82/LConn1 -- Transform83/LConn1 -- Transform84/LConn1 -- Transform85/LConn1 -- Transform86/LConn1 -- Transform87/LConn1 -- Transform88/LConn1 -- Transform89/LConn1 -- Transform9/LConn1 -- Transform90/LConn1 -- Transform91/LConn1 -- Transform92/LConn1 -- Transform93/LConn1 -- Transform94/LConn1 -- Transform95/LConn1 -- Transform96/LConn1 -- Transform97/LConn1 -- Transform98/LConn1 -- Transform99/LConn1 -- F1/RConn1
  Transform/RConn1 -- F/RConn1
  Transform9/RConn1 -- pan_cross_head_am_68_RIGID/LConn1
  Transform99/RConn1 -- instrument_ball_bearing_68_am_41_RIGID/LConn1
  Joint1_Ring_Spacers_28_RIGID/LConn1 -- Transform100/RConn1
  Transform101/RConn1 -- instrument_ball_bearing_68_am_46_RIGID/LConn1
  Transform102/RConn1 -- instrument_ball_bearing_68_am_47_RIGID/LConn1
  Transform103/RConn1 -- instrument_ball_bearing_68_am_48_RIGID/LConn1
  Transform104/RConn1 -- instrument_ball_bearing_68_am_53_RIGID/LConn1
  Joint1_Ring_Spacers_34_RIGID/LConn1 -- Transform105/RConn1
  Transform106/RConn1 -- instrument_ball_bearing_68_am_55_RIGID/LConn1
  Transform107/RConn1 -- instrument_ball_bearing_68_am_57_RIGID/LConn1
  Transform108/RConn1 -- hex_screw_am_6_RIGID/LConn1
  Transform10/RConn1 -- pan_cross_head_am_70_RIGID/LConn1
  Transform109/RConn1 -- instrument_ball_bearing_68_am_58_RIGID/LConn1
  Transform110/RConn1 -- hex_screw_am_22_RIGID/LConn1
  Transform111/RConn1 -- hex_nut_style_2_ams_2_RIGID/LConn1
  Transform112/RConn1 -- hex_screw_am_8_RIGID/LConn1
  Transform113/RConn1 -- instrument_ball_bearing_68_am_61_RIGID/LConn1
  Transform114/RConn1 -- hex_screw_am_24_RIGID/LConn1
  Transform115/RConn1 -- hex_screw_am_18_RIGID/LConn1
  Transform116/RConn1 -- instrument_ball_bearing_68_am_67_RIGID/LConn1
  Transform117/RConn1 -- instrument_ball_bearing_68_am_65_RIGID/LConn1
  Transform118/RConn1 -- hex_screw_am_10_RIGID/LConn1
  Transform11/RConn1 -- pan_cross_head_am_74_RIGID/LConn1
  Transform119/RConn1 -- hex_screw_am_11_RIGID/LConn1
  Transform120/RConn1 -- hex_screw_am_9_RIGID/LConn1
  Transform121/RConn1 -- hex_screw_am_13_RIGID/LConn1
  Transform122/RConn1 -- instrument_ball_bearing_68_am_60_RIGID/LConn1
  Transform123/RConn1 -- socket_set_screw_cone_point_am_1_RIGID/LConn1
  Transform124/RConn1 -- hex_screw_am_5_RIGID/LConn1
  Transform125/RConn1 -- hex_screw_am_14_RIGID/LConn1
  Transform126/RConn1 -- hex_screw_am_17_RIGID/LConn1
  Transform127/RConn1 -- hex_screw_am_15_RIGID/LConn1
  Transform128/RConn1 -- hex_screw_am_12_RIGID/LConn1
  Transform12/RConn1 -- pan_cross_head_am_77_RIGID/LConn1
  Transform129/RConn1 -- hex_screw_am_7_RIGID/LConn1
  Transform130/RConn1 -- hex_screw_am_16_RIGID/LConn1
  Transform131/RConn1 -- hex_screw_am_19_RIGID/LConn1
  Transform132/RConn1 -- hex_screw_am_20_RIGID/LConn1
  Transform133/RConn1 -- instrument_ball_bearing_68_am_59_RIGID/LConn1
  Transform134/RConn1 -- hex_screw_am_23_RIGID/LConn1
  Transform135/RConn1 -- instrument_ball_bearing_68_am_63_RIGID/LConn1
  Transform136/RConn1 -- instrument_ball_bearing_68_am_64_RIGID/LConn1
  Transform137/RConn1 -- instrument_ball_bearing_68_am_62_RIGID/LConn1
  Transform138/RConn1 -- instrument_ball_bearing_68_am_66_RIGID/LConn1
  Transform13/RConn1 -- pan_cross_head_am_69_RIGID/LConn1
  Transform139/RConn1 -- instrument_ball_bearing_68_am_73_RIGID/LConn1
  Transform140/RConn1 -- instrument_ball_bearing_68_am_69_RIGID/LConn1
  Transform141/RConn1 -- hex_screw_am_25_RIGID/LConn1
  Transform142/RConn1 -- instrument_ball_bearing_68_am_70_RIGID/LConn1
  Transform143/RConn1 -- instrument_ball_bearing_68_am_71_RIGID/LConn1
  Transform144/RConn1 -- instrument_ball_bearing_68_am_68_RIGID/LConn1
  Transform145/RConn1 -- instrument_ball_bearing_68_am_72_RIGID/LConn1
  Transform146/RConn1 -- hex_screw_am_29_RIGID/LConn1
  Transform147/RConn1 -- instrument_ball_bearing_68_am_76_RIGID/LConn1
  Transform148/RConn1 -- instrument_ball_bearing_68_am_77_RIGID/LConn1
  Transform14/RConn1 -- instrument_ball_bearing_68_am_92_RIGID/LConn1
  Transform149/RConn1 -- instrument_ball_bearing_68_am_79_RIGID/LConn1
  Transform150/RConn1 -- hex_screw_am_28_RIGID/LConn1
  Transform151/RConn1 -- instrument_ball_bearing_68_am_75_RIGID/LConn1
  Transform152/RConn1 -- instrument_ball_bearing_68_am_80_RIGID/LConn1
  Transform153/RConn1 -- instrument_ball_bearing_68_am_82_RIGID/LConn1
  Transform154/RConn1 -- instrument_ball_bearing_68_am_83_RIGID/LConn1
  Transform155/RConn1 -- instrument_ball_bearing_68_am_84_RIGID/LConn1
  Transform156/RConn1 -- instrument_ball_bearing_68_am_85_RIGID/LConn1
  Transform157/RConn1 -- instrument_ball_bearing_68_am_74_RIGID/LConn1
  Transform158/RConn1 -- hex_screw_am_27_RIGID/LConn1
  Transform15/RConn1 -- instrument_ball_bearing_68_am_95_RIGID/LConn1
  Transform159/RConn1 -- instrument_ball_bearing_68_am_87_RIGID/LConn1
  Transform160/RConn1 -- hex_screw_am_26_RIGID/LConn1
  Transform161/RConn1 -- instrument_ball_bearing_68_am_78_RIGID/LConn1
  Transform162/RConn1 -- instrument_ball_bearing_68_am_81_RIGID/LConn1
  Transform163/RConn1 -- instrument_ball_bearing_68_am_88_RIGID/LConn1
  Transform164/RConn1 -- instrument_ball_bearing_68_am_89_RIGID/LConn1
  Transform165/RConn1 -- instrument_ball_bearing_68_am_86_RIGID/LConn1
  Transform166/RConn1 -- pan_cross_head_am_44_RIGID/LConn1
  Transform167/RConn1 -- pan_cross_head_am_45_RIGID/LConn1
  Transform168/RConn1 -- instrument_ball_bearing_68_am_90_RIGID/LConn1
  Transform16/RConn1 -- instrument_ball_bearing_68_am_96_RIGID/LConn1
  Transform169/RConn1 -- pan_cross_head_am_46_RIGID/LConn1
  Transform170/RConn1 -- pan_cross_head_am_47_RIGID/LConn1
  Transform171/RConn1 -- pan_cross_head_am_48_RIGID/LConn1
  Transform172/RConn1 -- x15_1_CycloDisk_1_RIGID/LConn1
  Transform173/RConn1 -- hex_screw_am_3_RIGID/LConn1
  Joint1_Ring_Spacers_4_RIGID/LConn1 -- Transform174/RConn1
  Transform175/RConn1 -- instrument_ball_bearing_68_am_11_RIGID/LConn1
  Joint1_Eccentric_Shaft_1_RIGID/LConn1 -- Transform176/RConn1
  Joint1_Cyclo_Output_Shaft_1_RIGID/LConn1 -- Transform177/RConn1
  Joint1_Cover_1_RIGID/LConn1 -- Transform178/RConn1
  Transform17/RConn1 -- pan_cross_head_am_51_RIGID/LConn1
  Main_Basee_Joint1_1_RIGID/LConn1 -- Transform179/RConn1
  NEMA23_Bipolar_1_RIGID/LConn1 -- Transform180/RConn1
  Transform181/RConn1 -- formed_hex_screw_am_1_RIGID/LConn1
  Transform182/RConn1 -- User_Library_15x28x7_brg_2_RIGID/LConn1
  Transform183/RConn1 -- formed_hex_screw_am_6_RIGID/LConn1
  Transform184/RConn1 -- hex_screw_am_1_RIGID/LConn1
  Transform185/RConn1 -- instrument_ball_bearing_68_am_5_RIGID/LConn1
  Joint1_Ring_Spacers_7_RIGID/LConn1 -- Transform186/RConn1
  Transform187/RConn1 -- formed_hex_screw_am_4_RIGID/LConn1
  Joint1_Top_Cover_1_RIGID/LConn1 -- Transform188/RConn1
  Transform18/RConn1 -- pan_cross_head_am_58_RIGID/LConn1
  Transform189/RConn1 -- formed_hex_screw_am_5_RIGID/LConn1
  Transform190/RConn1 -- instrument_ball_bearing_68_am_4_RIGID/LConn1
  Transform191/RConn1 -- User_Library_15x28x7_brg_1_RIGID/LConn1
  Transform192/RConn1 -- x15_1_CycloDisk_2_RIGID/LConn1
  Joint1_Main_Case_1_RIGID/LConn1 -- Transform193/RConn1
  Transform194/RConn1 -- hex_screw_am_2_RIGID/LConn1
  Joint1_Ring_Spacers_3_RIGID/LConn1 -- Transform195/RConn1
  Transform196/RConn1 -- instrument_ball_bearing_68_am_6_RIGID/LConn1
  Joint1_Ring_Spacers_14_RIGID/LConn1 -- Transform197/RConn1
  Joint1_Ring_Spacers_17_RIGID/LConn1 -- Transform198/RConn1
  Transform1/RConn1 -- pan_cross_head_am_78_RIGID/LConn1
  Transform19/RConn1 -- pan_cross_head_am_60_RIGID/LConn1
  Joint1_Ring_Spacers_10_RIGID/LConn1 -- Transform199/RConn1
  Joint1_Ring_Spacers_11_RIGID/LConn1 -- Transform200/RConn1
  Transform201/RConn1 -- instrument_ball_bearing_68_am_20_RIGID/LConn1
  Transform202/RConn1 -- instrument_ball_bearing_68_am_22_RIGID/LConn1
  Transform203/RConn1 -- instrument_ball_bearing_68_am_24_RIGID/LConn1
  Transform204/RConn1 -- instrument_ball_bearing_68_am_14_RIGID/LConn1
  Transform205/RConn1 -- instrument_ball_bearing_68_am_18_RIGID/LConn1
  Joint1_Ring_Spacers_16_RIGID/LConn1 -- Transform206/RConn1
  Transform207/RConn1 -- instrument_ball_bearing_68_am_21_RIGID/LConn1
  Transform208/RConn1 -- instrument_ball_bearing_68_am_25_RIGID/LConn1
  Transform20/RConn1 -- pan_cross_head_am_55_RIGID/LConn1
  Transform209/RConn1 -- instrument_ball_bearing_68_am_23_RIGID/LConn1
  Joint1_Ring_Spacers_22_RIGID/LConn1 -- Transform210/RConn1
  Transform211/RConn1 -- instrument_ball_bearing_68_am_16_RIGID/LConn1
  Joint1_Ring_Spacers_12_RIGID/LConn1 -- Transform212/RConn1
  Joint1_Ring_Spacers_9_RIGID/LConn1 -- Transform213/RConn1
  Transform214/RConn1 -- instrument_ball_bearing_68_am_13_RIGID/LConn1
  Transform215/RConn1 -- instrument_ball_bearing_68_am_15_RIGID/LConn1
  Joint1_Ring_Spacers_13_RIGID/LConn1 -- Transform216/RConn1
  Transform217/RConn1 -- instrument_ball_bearing_68_am_19_RIGID/LConn1
  Transform218/RConn1 -- instrument_ball_bearing_68_am_12_RIGID/LConn1
  Transform21/RConn1 -- pan_cross_head_am_59_RIGID/LConn1
  Joint1_Ring_Spacers_8_RIGID/LConn1 -- Transform219/RConn1
  Transform220/RConn1 -- instrument_ball_bearing_68_am_17_RIGID/LConn1
  Joint1_Ring_Spacers_15_RIGID/LConn1 -- Transform221/RConn1
  Transform222/RConn1 -- instrument_ball_bearing_68_am_26_RIGID/LConn1
  Transform223/RConn1 -- instrument_ball_bearing_68_am_29_RIGID/LConn1
  Joint1_Ring_Spacers_20_RIGID/LConn1 -- Transform224/RConn1
  Transform225/RConn1 -- instrument_ball_bearing_68_am_32_RIGID/LConn1
  Transform226/RConn1 -- instrument_ball_bearing_68_am_33_RIGID/LConn1
  Transform227/RConn1 -- instrument_ball_bearing_68_am_28_RIGID/LConn1
  Joint1_Ring_Spacers_19_RIGID/LConn1 -- Transform228/RConn1
  Transform22/RConn1 -- hex_nut_style_1_am_5_RIGID/LConn1
  Transform229/RConn1 -- instrument_ball_bearing_68_am_31_RIGID/LConn1
  Joint1_Ring_Spacers_18_RIGID/LConn1 -- Transform230/RConn1
  Transform231/RConn1 -- instrument_ball_bearing_68_am_30_RIGID/LConn1
  Joint1_Ring_Spacers_21_RIGID/LConn1 -- Transform232/RConn1
  Transform233/RConn1 -- instrument_ball_bearing_68_am_27_RIGID/LConn1
  Transform234/RConn1 -- instrument_ball_bearing_68_am_34_RIGID/LConn1
  Joint1_Ring_Spacers_23_RIGID/LConn1 -- Transform235/RConn1
  Transform236/RConn1 -- instrument_ball_bearing_68_am_35_RIGID/LConn1
  Transform23/RConn1 -- pan_cross_head_am_50_RIGID/LConn1
  Transform24/RConn1 -- pan_cross_head_am_56_RIGID/LConn1
  Transform25/RConn1 -- instrument_ball_bearing_68_am_93_RIGID/LConn1
  Transform26/RConn1 -- instrument_ball_bearing_68_am_101_RIGID/LConn1
  Transform27/RConn1 -- instrument_ball_bearing_68_am_102_RIGID/LConn1
  Transform28/RConn1 -- pan_cross_head_am_54_RIGID/LConn1
  Transform2/RConn1 -- pan_cross_head_am_67_RIGID/LConn1
  Transform29/RConn1 -- instrument_ball_bearing_68_am_97_RIGID/LConn1
  Transform30/RConn1 -- instrument_ball_bearing_68_am_98_RIGID/LConn1
  Transform31/RConn1 -- instrument_ball_bearing_68_am_91_RIGID/LConn1
  Transform32/RConn1 -- pan_cross_head_am_53_RIGID/LConn1
  Transform33/RConn1 -- pan_cross_head_am_52_RIGID/LConn1
  Transform34/RConn1 -- pan_cross_head_am_57_RIGID/LConn1
  Transform35/RConn1 -- pan_cross_head_am_49_RIGID/LConn1
  Transform36/RConn1 -- instrument_ball_bearing_68_am_94_RIGID/LConn1
  Transform37/RConn1 -- instrument_ball_bearing_68_am_99_RIGID/LConn1
  Transform38/RConn1 -- hex_nut_style_1_am_3_RIGID/LConn1
  Transform3/RConn1 -- pan_cross_head_am_71_RIGID/LConn1
  Transform39/RConn1 -- hex_nut_style_1_am_4_RIGID/LConn1
  Transform40/RConn1 -- hex_nut_style_1_am_6_RIGID/LConn1
  Transform41/RConn1 -- instrument_ball_bearing_68_am_103_RIGID/LConn1
  Transform42/RConn1 -- hex_nut_style_1_am_2_RIGID/LConn1
  Transform43/RConn1 -- instrument_ball_bearing_68_am_100_RIGID/LConn1
  Transform44/RConn1 -- hex_nut_style_1_am_12_RIGID/LConn1
  Transform45/RConn1 -- formed_hex_screw_am_19_RIGID/LConn1
  Transform46/RConn1 -- hex_nut_style_1_am_13_RIGID/LConn1
  Transform47/RConn1 -- hex_nut_style_1_am_14_RIGID/LConn1
  Transform48/RConn1 -- formed_hex_screw_am_11_RIGID/LConn1
  Transform4/RConn1 -- pan_cross_head_am_72_RIGID/LConn1
  Transform49/RConn1 -- formed_hex_screw_am_16_RIGID/LConn1
  Transform50/RConn1 -- formed_hex_screw_am_17_RIGID/LConn1
  Transform51/RConn1 -- formed_hex_screw_am_13_RIGID/LConn1
  Transform52/RConn1 -- hex_nut_style_1_am_9_RIGID/LConn1
  Transform53/RConn1 -- hex_nut_style_1_am_11_RIGID/LConn1
  Ball_Bearing_Retainer_1_RIGID/LConn1 -- Transform54/RConn1
  Transform55/RConn1 -- pan_cross_head_am_61_RIGID/LConn1
  Transform56/RConn1 -- hex_nut_style_1_am_7_RIGID/LConn1
  Transform57/RConn1 -- formed_hex_screw_am_9_RIGID/LConn1
  Transform58/RConn1 -- pan_cross_head_am_62_RIGID/LConn1
  Transform5/RConn1 -- pan_cross_head_am_73_RIGID/LConn1
  Transform59/RConn1 -- pan_cross_head_am_63_RIGID/LConn1
  Transform60/RConn1 -- hex_nut_style_1_am_8_RIGID/LConn1
  Transform61/RConn1 -- formed_hex_screw_am_15_RIGID/LConn1
  Transform62/RConn1 -- formed_hex_screw_am_10_RIGID/LConn1
  Transform63/RConn1 -- formed_hex_screw_am_12_RIGID/LConn1
  Transform64/RConn1 -- formed_hex_screw_am_18_RIGID/LConn1
  Transform65/RConn1 -- formed_hex_screw_am_20_RIGID/LConn1
  Transform66/RConn1 -- formed_hex_screw_am_24_RIGID/LConn1
  Transform67/RConn1 -- instrument_ball_bearing_68_am_104_RIGID/LConn1
  Transform68/RConn1 -- instrument_ball_bearing_68_am_105_RIGID/LConn1
  Transform6/RConn1 -- pan_cross_head_am_75_RIGID/LConn1
  Transform69/RConn1 -- hex_nut_jam_am_3_RIGID/LConn1
  Shaftt_Blocker_1_RIGID/LConn1 -- Transform70/RConn1
  Transform71/RConn1 -- formed_hex_screw_am_22_RIGID/LConn1
  Transform72/RConn1 -- pan_cross_head_am_66_RIGID/LConn1
  Transform73/RConn1 -- pan_cross_head_am_65_RIGID/LConn1
  Transform74/RConn1 -- pan_cross_head_am_64_RIGID/LConn1
  Joint1_Ring_Spacers_27_RIGID/LConn1 -- Transform75/RConn1
  Transform76/RConn1 -- instrument_ball_bearing_68_am_38_RIGID/LConn1
  Transform77/RConn1 -- instrument_ball_bearing_68_am_43_RIGID/LConn1
  Joint1_Ring_Spacers_31_RIGID/LConn1 -- Transform78/RConn1
  Transform7/RConn1 -- x36_Teeth_Pulley_1_RIGID/LConn1
  Transform79/RConn1 -- instrument_ball_bearing_68_am_44_RIGID/LConn1
  Transform80/RConn1 -- instrument_ball_bearing_68_am_52_RIGID/LConn1
  Transform81/RConn1 -- instrument_ball_bearing_68_am_37_RIGID/LConn1
  Transform82/RConn1 -- instrument_ball_bearing_68_am_54_RIGID/LConn1
  Transform83/RConn1 -- instrument_ball_bearing_68_am_56_RIGID/LConn1
  Joint1_Ring_Spacers_36_RIGID/LConn1 -- Transform84/RConn1
  Joint1_Ring_Spacers_24_RIGID/LConn1 -- Transform85/RConn1
  Transform86/RConn1 -- instrument_ball_bearing_68_am_45_RIGID/LConn1
  Joint1_Ring_Spacers_32_RIGID/LConn1 -- Transform87/RConn1
  Transform88/RConn1 -- instrument_ball_bearing_68_am_36_RIGID/LConn1
  Transform8/RConn1 -- pan_cross_head_am_76_RIGID/LConn1
  Transform89/RConn1 -- instrument_ball_bearing_68_am_49_RIGID/LConn1
  Joint1_Ring_Spacers_33_RIGID/LConn1 -- Transform90/RConn1
  Joint1_Ring_Spacers_35_RIGID/LConn1 -- Transform91/RConn1
  Transform92/RConn1 -- instrument_ball_bearing_68_am_42_RIGID/LConn1
  Transform93/RConn1 -- instrument_ball_bearing_68_am_39_RIGID/LConn1
  Joint1_Ring_Spacers_29_RIGID/LConn1 -- Transform94/RConn1
  Joint1_Ring_Spacers_30_RIGID/LConn1 -- Transform95/RConn1
  Joint1_Ring_Spacers_25_RIGID/LConn1 -- Transform96/RConn1
  Joint1_Ring_Spacers_26_RIGID/LConn1 -- Transform97/RConn1
  Transform98/RConn1 -- instrument_ball_bearing_68_am_40_RIGID/LConn1
